simulink model "Demo_CarRealTime2D_cs"  (R2014b)
settings: Solver=ode5  SolverMode=SingleTasking  StartTime=0.0  StopTime=inf  FixedStep=1/1000  RelTol=1e-3
PreLoadFcn:
  | mbxruntime.callbacks.PreLoadFcn(bdroot);
  | check_NUTS_defined;
  | assignin('base',['model_closed_' bdroot],false);
  | addpath('../includes_AEBS');
PostLoadFcn:
  | mbxruntime.callbacks.PostLoadFcn(bdroot);
InitFcn:
  | mbxruntime.callbacks.InitFcn(bdroot);
StartFcn:
  | mbxruntime.callbacks.StartFcn(bdroot);
StopFcn:
  | mbxruntime.callbacks.StopFcn(bdroot);;
  | 
model workspace: external: MAT-File .\Demo_CarRealTime2D_cs_hws.mat (data not in the file)
undefined symbols (not defined in the file or in its folder): Driver_Demands, mbxruntime, tabledata, vicrt_initcallback, vicrt_initmexcallback, vicrt_simulationmanager, warningInitialVelocity, x0
undefined symbols (not defined in the file): Demo_CarRealTime2D_cs_007c1c37f387f47f, Demo_CarRealTime2D_cs_085a64a83ba38cec, Demo_CarRealTime2D_cs_0a7f542d3fc7ab9f, Demo_CarRealTime2D_cs_0d7c72cfaa56dff7, Demo_CarRealTime2D_cs_0de07b35068e3828, Demo_CarRealTime2D_cs_17f4d381375cce95, Demo_CarRealTime2D_cs_1db40a09b08215a9, Demo_CarRealTime2D_cs_2bfa3850c176687b, Demo_CarRealTime2D_cs_35a34f1ba6ce4a22, Demo_CarRealTime2D_cs_378cc77e08d643fb, Demo_CarRealTime2D_cs_409b5c3befba0000, Demo_CarRealTime2D_cs_42628ca5bb62d2f3, Demo_CarRealTime2D_cs_56554a2db408a7f8, Demo_CarRealTime2D_cs_59527455249d7429, Demo_CarRealTime2D_cs_5983ee1b8112afac, Demo_CarRealTime2D_cs_5b5ebcf3ed7bf8e6, Demo_CarRealTime2D_cs_63cbe7fbe16cd5d9, Demo_CarRealTime2D_cs_6e17b9adbf989abf, Demo_CarRealTime2D_cs_6f662a34e5d9a196, Demo_CarRealTime2D_cs_75c4ee8892821e19, Demo_CarRealTime2D_cs_7c64486355814be2, Demo_CarRealTime2D_cs_849809550a2230ef, Demo_CarRealTime2D_cs_87f899bcbe16d8f5, Demo_CarRealTime2D_cs_8e7b50dac25b68a2, Demo_CarRealTime2D_cs_94938e5260f139b3, Demo_CarRealTime2D_cs_983acc940698d1d1, Demo_CarRealTime2D_cs_9d554c72797f76fd, Demo_CarRealTime2D_cs_9d747ee2f15c057f, Demo_CarRealTime2D_cs_ad62a2084d31e898, Demo_CarRealTime2D_cs_b56c8c5f000d30f0, Demo_CarRealTime2D_cs_b95f1b7356e926cc, Demo_CarRealTime2D_cs_BMW_X5_1_Path_pathUniqueID, Demo_CarRealTime2D_cs_BMW_Z3_2_Dynamics_Empty_STATE_BMW_Z3_2_x0, Demo_CarRealTime2D_cs_BMW_Z3_2_Dynamics_Empty_STATE_BMW_Z3_2_y0, Demo_CarRealTime2D_cs_BMW_Z3_2_Dynamics_Empty_STATE_BMW_Z3_2_z0, Demo_CarRealTime2D_cs_BMW_Z3_Path_pathUniqueID, Demo_CarRealTime2D_cs_BMW_Z3_SpeedProfile_speedProfileUniqueID, Demo_CarRealTime2D_cs_c8847ab2e5633224, Demo_CarRealTime2D_cs_c9a0d701286b93fb, Demo_CarRealTime2D_cs_ce758cae7dd1b283, Demo_CarRealTime2D_cs_CrossingPedestrian_Path_pathUniqueID, Demo_CarRealTime2D_cs_CuttingInVehicle_Path_pathUniqueID, Demo_CarRealTime2D_cs_d901ab1c1d2e40bc, Demo_CarRealTime2D_cs_dff70430e5a00a86, Demo_CarRealTime2D_cs_ef038a4f619ad32e, Demo_CarRealTime2D_cs_Female_OverweightAni_1_Path_pathUniqueID, Demo_CarRealTime2D_cs_Ford_Fiesta_1_Path_pathUniqueID, Demo_CarRealTime2D_cs_Ford_FocusWagon_Path_pathUniqueID, Demo_CarRealTime2D_cs_Sphere_1_Dynamics_Empty_STATE_Sphere_1_x0, Demo_CarRealTime2D_cs_Sphere_1_Dynamics_Empty_STATE_Sphere_1_y0, Demo_CarRealTime2D_cs_Sphere_1_Dynamics_Empty_STATE_Sphere_1_z0, WheelL0, WheelL1, WheelR0, WheelR1
libraries: PreScanSimulinkLibrary x15, simulink x15, simulink_extras x15, PreScanUsefulBlocks x2, dspsigops x1
(part 15 of 17)

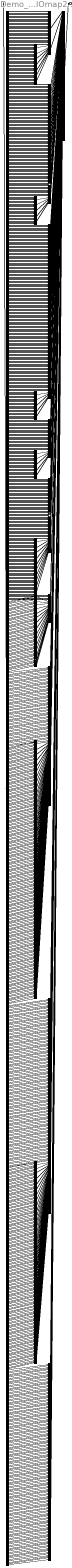
== system Demo_CarRealTime2D_cs/HostVehicle/Dynamics_UserSpecified/VI-CarRealTime/Output_Bus/IOmap2bus ==
  In : Inport
  Actual_Tread_Speed : BusCreator
  Aggregate_Force_At_Wheel : BusCreator
  Alpha : BusCreator
  Animator_Widget : BusCreator  Inputs=2
  Auxiliary_Roll_Force : BusCreator
  Auxiliary_Roll_Force_at_element : BusCreator  Inputs=2
  Auxiliary_Roll_deformation_at_element : BusCreator  Inputs=2
  Brake : BusCreator  Inputs=7
  Brake_Moment : BusCreator
  Caster_Angle : BusCreator  Inputs=2
  Chamber_Pressure : BusCreator
  Contact_Patch_Global_X : BusCreator
  Contact_Patch_Global_Y : BusCreator
  Contact_Patch_Global_Z : BusCreator
  Contact_Patch_Global_dZdX : BusCreator
  Contact_Patch_Global_dZdY : BusCreator
  Damper : BusCreator  Inputs=5
  Demux : Demux  Outputs=1108
  Drive_Moment : BusCreator
  Effective_Closing_Speed : BusCreator
  Effective_Penetration : BusCreator
  Effective_Rolling_Radius : BusCreator
  Equivalent_Tread_Speed : BusCreator
  Euler_Roll : BusCreator
  External_Friction_Scale_Factor : BusCreator
  Force_At_Bumper : BusCreator
  Force_At_Bumper1 : BusCreator
  Force_At_Damper : BusCreator
  Force_At_Spring : BusCreator
  Force_At_Wheel{,1..3} (4 alike) : BusCreator
  Force_Aux_At_Wheel : BusCreator
  Global_Omega_X : BusCreator
  Global_Omega_Y : BusCreator
  Global_Omega_Z : BusCreator
  Global_Vx : BusCreator
  Global_Vy : BusCreator
  Global_Vz : BusCreator
  Global_X : BusCreator
  Global_Y : BusCreator
  Global_Z : BusCreator
  Ground_Surface_Contact_Patch_Vx : BusCreator
  Ground_Surface_Contact_Patch_Vy : BusCreator
  Ground_Surface_Force_X : BusCreator
  Ground_Surface_Force_Y : BusCreator
  Ground_Surface_Force_Z : BusCreator
  Ground_Surface_Gyroscopic_Moment : BusCreator
  Ground_Surface_Kappa_Fy : BusCreator
  Ground_Surface_Moment_X : BusCreator
  Ground_Surface_Moment_Y : BusCreator
  Ground_Surface_Moment_Z : BusCreator
  Ground_Surface_Peak_Friction_X : BusCreator
  Ground_Surface_Peak_Friction_Y : BusCreator
  Ground_Surface_Residual_Torque : BusCreator
  Ground_Surface_Wheel_Center_Vx : BusCreator
  Gyro : BusCreator  Inputs=10
  Hook_rear : BusCreator  Inputs=18
  Hub_Carrier_Force_Global_X : BusCreator
  Hub_Carrier_Force_Global_Y : BusCreator
  Hub_Carrier_Force_Global_Z : BusCreator
  Hub_Carrier_Force_Local_X : BusCreator
  Hub_Carrier_Force_Local_Y : BusCreator
  Hub_Carrier_Force_Local_Z : BusCreator
  Hub_Carrier_Moment_Global_X : BusCreator
  Hub_Carrier_Moment_Global_Y : BusCreator
  Hub_Carrier_Moment_Global_Z : BusCreator
  Hub_Carrier_Moment_Local_X : BusCreator
  Hub_Carrier_Moment_Local_Y : BusCreator
  Hub_Carrier_Moment_Local_Z : BusCreator
  Hub_Carrier_Omega_X : BusCreator
  Hub_Carrier_Omega_Y : BusCreator
  Hub_Carrier_Omega_Z : BusCreator
  Hub_Carrier_Vx : BusCreator
  Hub_Carrier_Vy : BusCreator
  Hub_Carrier_Vz : BusCreator
  Inclination : BusCreator
  Inst_Stiff_Deflection : BusCreator
  Inst_Stiff_Force : BusCreator
  Jounce{,1..4} (5 alike) : BusCreator
  Jounce_Acceleration{,1..4} (5 alike) : BusCreator
  Jounce_Bumper : BusCreator  Inputs=5
  Jounce_Rate{,1..4} (5 alike) : BusCreator
  Kingpin_Moment : BusCreator  Inputs=1
  Kingpin_Moment1 : BusCreator  Inputs=2
  Lateral_Relaxation_Length : BusCreator
  Lateral_Slip_With_Lag : BusCreator
  Lateral_Slip_Without_Lag : BusCreator
  Loaded_Radius : BusCreator
  Locked_Damper_Moment : BusCreator
  Locked_Moment : BusCreator
  Locked_Spring_Moment : BusCreator
  Locked_Switch : BusCreator
  Lockup_Rotation : BusCreator
  Longitudinal_Relaxation_Length : BusCreator
  Longitudinal_Slip_With_Lag : BusCreator
  Longitudinal_Slip_Without_Lag : BusCreator
  Moment_Arm_Of_Fx : BusCreator
  Omega : BusCreator
  OutputBus : BusCreator  Inputs=92
  PID_CW_At_Spring : BusCreator
  PID_PH_At_Spring : BusCreator
  PID_RH_At_Spring : BusCreator
  Phi : BusCreator
  Pitch : BusCreator
  Pneumatic_Trail : BusCreator
  Psi : BusCreator
  Rebound_Bumper : BusCreator  Inputs=5
  Roll : BusCreator  Inputs=2
  Rotation : BusCreator
  Sensor : BusCreator  Inputs=16
  Side_View_Angle : BusCreator
  Spindle_Steer : BusCreator
  Spring : BusCreator  Inputs=10
  Steering_Instant_Axis_Rotation : BusCreator  Inputs=2
  Steering_System : BusCreator  Inputs=6
  Suspension : BusCreator  Inputs=14
  System : BusCreator
  System_Mass_Center : BusCreator  Inputs=13
  Theta : BusCreator
  TieRod_Force_Left : BusCreator  Inputs=3
  TieRod_Force_Right : BusCreator  Inputs=3
  Tire : BusCreator  Inputs=46
  User_Input_Contact_Patch_Global_Z_Perturbation : BusCreator
  Vehicle : BusCreator  Inputs=46
  Vehicle_States : BusCreator  Inputs=20
  Wheel : BusCreator  Inputs=37
  Yaw : BusCreator
  aero_forces : BusCreator  Inputs=24
  base_acceleration : BusCreator
  base_deformation : BusCreator
  base_velocity : BusCreator
  bul_jounce_stop_data : BusCreator  Inputs=6
  bul_rebound_stop_data : BusCreator  Inputs=6
  bur_jounce_stop_data : BusCreator  Inputs=6
  bur_rebound_stop_data : BusCreator  Inputs=6
  bus_dmp_jounce_stop_data : BusCreator  Inputs=6
  bus_ins_jounce_stop_data : BusCreator  Inputs=6
  bus_roll_dmp_jounce_stop_data : BusCreator  Inputs=6
  bus_spr_jounce_stop_data : BusCreator  Inputs=6
  chassis_accelerations : BusCreator  Inputs=6
  chassis_displacements : BusCreator  Inputs=9
  chassis_velocities : BusCreator  Inputs=6
  clutch : BusCreator  Inputs=2
  condition_sensors : BusCreator  Inputs=1
  cp_force_lateralFL : BusCreator  Inputs=3
  cp_force_lateralFR : BusCreator  Inputs=3
  cp_force_lateralRL : BusCreator  Inputs=3
  cp_force_lateralRR : BusCreator  Inputs=3
  cp_force_longitudinalFL : BusCreator  Inputs=3
  cp_force_longitudinalFR : BusCreator  Inputs=3
  cp_force_longitudinalRL : BusCreator  Inputs=3
  cp_force_longitudinalRR : BusCreator  Inputs=3
  cp_force_normalFL : BusCreator  Inputs=3
  cp_force_normalFR : BusCreator  Inputs=3
  cp_force_normalRL : BusCreator  Inputs=3
  cp_force_normalRR : BusCreator  Inputs=3
  cross_weight : BusCreator
  dal_ride_damper_data : BusCreator
  dar_ride_damper_data : BusCreator
  das_ride_damper_data : BusCreator  Inputs=6
  das_roll_damper_data : BusCreator  Inputs=8
  das_third_damper_data : BusCreator  Inputs=6
  differential_speeds : BusCreator  Inputs=6
  differential_torques : BusCreator  Inputs=6
  driver_demands : BusCreator  Inputs=7
  driving_machine_monitor : BusCreator  Inputs=9
  engine : BusCreator  Inputs=7
  fuel_consumption : BusCreator
  ges_chassis_XFORM : BusCreator  Inputs=6
  ges_hub_XFORMFL : BusCreator  Inputs=6
  ges_hub_XFORMFR : BusCreator  Inputs=6
  ges_hub_XFORMRL : BusCreator  Inputs=6
  ges_hub_XFORMRR : BusCreator  Inputs=6
  hub2cp_XFORMFL : BusCreator  Inputs=3
  hub2cp_XFORMFR : BusCreator  Inputs=3
  hub2cp_XFORMRL : BusCreator  Inputs=3
  hub2cp_XFORMRR : BusCreator  Inputs=3
  hub_center_accx : BusCreator
  hub_center_accy : BusCreator
  hub_center_accz : BusCreator
  ins_inerter_data : BusCreator  Inputs=10
  jfs_torsional_stiffness_data : BusCreator  Inputs=12
  nsl_ride_spring_data : BusCreator  Inputs=6
  nsr_ride_spring_data : BusCreator  Inputs=6
  nss_ride_spring_data : BusCreator  Inputs=10
  res_dmp_rebound_stop_data : BusCreator  Inputs=6
  res_ins_rebound_stop_data : BusCreator  Inputs=6
  res_roll_dmp_rebound_stop_data : BusCreator  Inputs=6
  res_spr_rebound_stop_data : BusCreator  Inputs=6
  rhl_front_setup_sensor_data : BusCreator  Inputs=1
  rhr_front_setup_sensor_data : BusCreator  Inputs=1
  rhs_rear_setup_sensor_data : BusCreator  Inputs=1
  til_wheel_tire_forces : BusCreator  Inputs=18
  til_wheel_tire_kinematics : BusCreator  Inputs=9
  til_wheel_tire_rolling_states : BusCreator  Inputs=9
  tir_wheel_tire_forces : BusCreator  Inputs=18
  tir_wheel_tire_kinematics : BusCreator  Inputs=9
  tir_wheel_tire_rolling_states : BusCreator  Inputs=9
  transmission : BusCreator
  ues_third_spring_data : BusCreator  Inputs=6
  upright_accelerometer : BusCreator
  wheel_angles : BusCreator  Inputs=12
  wheel_center_dispx : BusCreator
  wheel_center_dispy : BusCreator
  wheel_center_dispz : BusCreator
  whl_front_wheel_XFORM : BusCreator  Inputs=9
  whl_rear_wheel_XFORM : BusCreator  Inputs=9
  whl_twin_rear_wheel_XFORM : BusCreator  Inputs=9
  whr_front_wheel_XFORM : BusCreator  Inputs=9
  whr_rear_wheel_XFORM : BusCreator  Inputs=9
  whr_twin_rear_wheel_XFORM : BusCreator  Inputs=9
  Out : Outport
  wires:
  Demux/1108 -> cp_force_normalRR/3  "Z"
  Demux/1107 -> cp_force_normalRR/2  "Y"
  Demux/1106 -> cp_force_normalRR/1  "X"
  cp_force_normalRR/1 -> OutputBus/92  "cp_force_normalRR"
  Demux/1105 -> cp_force_lateralRR/3  "Z"
  Demux/1104 -> cp_force_lateralRR/2  "Y"
  Demux/1103 -> cp_force_lateralRR/1  "X"
  cp_force_lateralRR/1 -> OutputBus/91  "cp_force_lateralRR"
  Demux/1102 -> cp_force_longitudinalRR/3  "Z"
  Demux/1101 -> cp_force_longitudinalRR/2  "Y"
  Demux/1100 -> cp_force_longitudinalRR/1  "X"
  cp_force_longitudinalRR/1 -> OutputBus/90  "cp_force_longitudinalRR"
  Demux/1099 -> hub2cp_XFORMRR/3  "Z"
  Demux/1098 -> hub2cp_XFORMRR/2  "Y"
  Demux/1097 -> hub2cp_XFORMRR/1  "X"
  hub2cp_XFORMRR/1 -> OutputBus/89  "hub2cp_XFORMRR"
  Demux/1096 -> ges_hub_XFORMRR/6  "Phi"
  Demux/1095 -> ges_hub_XFORMRR/5  "Theta"
  Demux/1094 -> ges_hub_XFORMRR/4  "Psi"
  Demux/1093 -> ges_hub_XFORMRR/3  "Z"
  Demux/1092 -> ges_hub_XFORMRR/2  "Y"
  Demux/1091 -> ges_hub_XFORMRR/1  "X"
  ges_hub_XFORMRR/1 -> OutputBus/88  "ges_hub_XFORMRR"
  Demux/1090 -> cp_force_normalRL/3  "Z"
  Demux/1089 -> cp_force_normalRL/2  "Y"
  Demux/1088 -> cp_force_normalRL/1  "X"
  cp_force_normalRL/1 -> OutputBus/87  "cp_force_normalRL"
  Demux/1087 -> cp_force_lateralRL/3  "Z"
  Demux/1086 -> cp_force_lateralRL/2  "Y"
  Demux/1085 -> cp_force_lateralRL/1  "X"
  cp_force_lateralRL/1 -> OutputBus/86  "cp_force_lateralRL"
  Demux/1084 -> cp_force_longitudinalRL/3  "Z"
  Demux/1083 -> cp_force_longitudinalRL/2  "Y"
  Demux/1082 -> cp_force_longitudinalRL/1  "X"
  cp_force_longitudinalRL/1 -> OutputBus/85  "cp_force_longitudinalRL"
  Demux/1081 -> hub2cp_XFORMRL/3  "Z"
  Demux/1080 -> hub2cp_XFORMRL/2  "Y"
  Demux/1079 -> hub2cp_XFORMRL/1  "X"
  hub2cp_XFORMRL/1 -> OutputBus/84  "hub2cp_XFORMRL"
  Demux/1078 -> ges_hub_XFORMRL/6  "Phi"
  Demux/1077 -> ges_hub_XFORMRL/5  "Theta"
  Demux/1076 -> ges_hub_XFORMRL/4  "Psi"
  Demux/1075 -> ges_hub_XFORMRL/3  "Z"
  Demux/1074 -> ges_hub_XFORMRL/2  "Y"
  Demux/1073 -> ges_hub_XFORMRL/1  "X"
  ges_hub_XFORMRL/1 -> OutputBus/83  "ges_hub_XFORMRL"
  Demux/1072 -> cp_force_normalFR/3  "Z"
  Demux/1071 -> cp_force_normalFR/2  "Y"
  Demux/1070 -> cp_force_normalFR/1  "X"
  cp_force_normalFR/1 -> OutputBus/82  "cp_force_normalFR"
  Demux/1069 -> cp_force_lateralFR/3  "Z"
  Demux/1068 -> cp_force_lateralFR/2  "Y"
  Demux/1067 -> cp_force_lateralFR/1  "X"
  cp_force_lateralFR/1 -> OutputBus/81  "cp_force_lateralFR"
  Demux/1066 -> cp_force_longitudinalFR/3  "Z"
  Demux/1065 -> cp_force_longitudinalFR/2  "Y"
  Demux/1064 -> cp_force_longitudinalFR/1  "X"
  cp_force_longitudinalFR/1 -> OutputBus/80  "cp_force_longitudinalFR"
  Demux/1063 -> hub2cp_XFORMFR/3  "Z"
  Demux/1062 -> hub2cp_XFORMFR/2  "Y"
  Demux/1061 -> hub2cp_XFORMFR/1  "X"
  hub2cp_XFORMFR/1 -> OutputBus/79  "hub2cp_XFORMFR"
  Demux/1060 -> ges_hub_XFORMFR/6  "Phi"
  Demux/1059 -> ges_hub_XFORMFR/5  "Theta"
  Demux/1058 -> ges_hub_XFORMFR/4  "Psi"
  Demux/1057 -> ges_hub_XFORMFR/3  "Z"
  Demux/1056 -> ges_hub_XFORMFR/2  "Y"
  Demux/1055 -> ges_hub_XFORMFR/1  "X"
  ges_hub_XFORMFR/1 -> OutputBus/78  "ges_hub_XFORMFR"
  Demux/1054 -> cp_force_normalFL/3  "Z"
  Demux/1053 -> cp_force_normalFL/2  "Y"
  Demux/1052 -> cp_force_normalFL/1  "X"
  cp_force_normalFL/1 -> OutputBus/77  "cp_force_normalFL"
  Demux/1051 -> cp_force_lateralFL/3  "Z"
  Demux/1050 -> cp_force_lateralFL/2  "Y"
  Demux/1049 -> cp_force_lateralFL/1  "X"
  cp_force_lateralFL/1 -> OutputBus/76  "cp_force_lateralFL"
  Demux/1048 -> cp_force_longitudinalFL/3  "Z"
  Demux/1047 -> cp_force_longitudinalFL/2  "Y"
  Demux/1046 -> cp_force_longitudinalFL/1  "X"
  cp_force_longitudinalFL/1 -> OutputBus/75  "cp_force_longitudinalFL"
  Demux/1045 -> hub2cp_XFORMFL/3  "Z"
  Demux/1044 -> hub2cp_XFORMFL/2  "Y"
  Demux/1043 -> hub2cp_XFORMFL/1  "X"
  hub2cp_XFORMFL/1 -> OutputBus/74  "hub2cp_XFORMFL"
  Demux/1042 -> ges_hub_XFORMFL/6  "Phi"
  Demux/1041 -> ges_hub_XFORMFL/5  "Theta"
  Demux/1040 -> ges_hub_XFORMFL/4  "Psi"
  Demux/1039 -> ges_hub_XFORMFL/3  "Z"
  Demux/1038 -> ges_hub_XFORMFL/2  "Y"
  Demux/1037 -> ges_hub_XFORMFL/1  "X"
  ges_hub_XFORMFL/1 -> OutputBus/73  "ges_hub_XFORMFL"
  Demux/1036 -> Animator_Widget/2  "engine_rpm"
  Demux/1035 -> Animator_Widget/1  "longitudinal_speed"
  Animator_Widget/1 -> OutputBus/72  "Animator_Widget"
  Demux/1034 -> whr_twin_rear_wheel_XFORM/9  "Z"
  Demux/1033 -> whr_twin_rear_wheel_XFORM/8  "Y"
  Demux/1032 -> whr_twin_rear_wheel_XFORM/7  "X"
  Demux/1031 -> whr_twin_rear_wheel_XFORM/6  "Theta"
  Demux/1030 -> whr_twin_rear_wheel_XFORM/5  "Psi"
  Demux/1029 -> whr_twin_rear_wheel_XFORM/4  "Phi"
  Demux/1028 -> whr_twin_rear_wheel_XFORM/3  "FZ"
  Demux/1027 -> whr_twin_rear_wheel_XFORM/2  "FY"
  Demux/1026 -> whr_twin_rear_wheel_XFORM/1  "FX"
  whr_twin_rear_wheel_XFORM/1 -> OutputBus/71  "whr_twin_rear_wheel_XFORM"
  Demux/1025 -> whr_rear_wheel_XFORM/9  "Z"
  Demux/1024 -> whr_rear_wheel_XFORM/8  "Y"
  Demux/1023 -> whr_rear_wheel_XFORM/7  "X"
  Demux/1022 -> whr_rear_wheel_XFORM/6  "Theta"
  Demux/1021 -> whr_rear_wheel_XFORM/5  "Psi"
  Demux/1020 -> whr_rear_wheel_XFORM/4  "Phi"
  Demux/1019 -> whr_rear_wheel_XFORM/3  "FZ"
  Demux/1018 -> whr_rear_wheel_XFORM/2  "FY"
  Demux/1017 -> whr_rear_wheel_XFORM/1  "FX"
  whr_rear_wheel_XFORM/1 -> OutputBus/70  "whr_rear_wheel_XFORM"
  Demux/1016 -> whr_front_wheel_XFORM/9  "Z"
  Demux/1015 -> whr_front_wheel_XFORM/8  "Y"
  Demux/1014 -> whr_front_wheel_XFORM/7  "X"
  Demux/1013 -> whr_front_wheel_XFORM/6  "Theta"
  Demux/1012 -> whr_front_wheel_XFORM/5  "Psi"
  Demux/1011 -> whr_front_wheel_XFORM/4  "Phi"
  Demux/1010 -> whr_front_wheel_XFORM/3  "FZ"
  Demux/1009 -> whr_front_wheel_XFORM/2  "FY"
  Demux/1008 -> whr_front_wheel_XFORM/1  "FX"
  whr_front_wheel_XFORM/1 -> OutputBus/69  "whr_front_wheel_XFORM"
  Demux/1007 -> whl_twin_rear_wheel_XFORM/9  "Z"
  Demux/1006 -> whl_twin_rear_wheel_XFORM/8  "Y"
  Demux/1005 -> whl_twin_rear_wheel_XFORM/7  "X"
  Demux/1004 -> whl_twin_rear_wheel_XFORM/6  "Theta"
  Demux/1003 -> whl_twin_rear_wheel_XFORM/5  "Psi"
  Demux/1002 -> whl_twin_rear_wheel_XFORM/4  "Phi"
  Demux/1001 -> whl_twin_rear_wheel_XFORM/3  "FZ"
  Demux/1000 -> whl_twin_rear_wheel_XFORM/2  "FY"
  Demux/999 -> whl_twin_rear_wheel_XFORM/1  "FX"
  whl_twin_rear_wheel_XFORM/1 -> OutputBus/68  "whl_twin_rear_wheel_XFORM"
  Demux/998 -> whl_rear_wheel_XFORM/9  "Z"
  Demux/997 -> whl_rear_wheel_XFORM/8  "Y"
  Demux/996 -> whl_rear_wheel_XFORM/7  "X"
  Demux/995 -> whl_rear_wheel_XFORM/6  "Theta"
  Demux/994 -> whl_rear_wheel_XFORM/5  "Psi"
  Demux/993 -> whl_rear_wheel_XFORM/4  "Phi"
  Demux/992 -> whl_rear_wheel_XFORM/3  "FZ"
  Demux/991 -> whl_rear_wheel_XFORM/2  "FY"
  Demux/990 -> whl_rear_wheel_XFORM/1  "FX"
  whl_rear_wheel_XFORM/1 -> OutputBus/67  "whl_rear_wheel_XFORM"
  Demux/989 -> whl_front_wheel_XFORM/9  "Z"
  Demux/988 -> whl_front_wheel_XFORM/8  "Y"
  Demux/987 -> whl_front_wheel_XFORM/7  "X"
  Demux/986 -> whl_front_wheel_XFORM/6  "Theta"
  Demux/985 -> whl_front_wheel_XFORM/5  "Psi"
  Demux/984 -> whl_front_wheel_XFORM/4  "Phi"
  Demux/983 -> whl_front_wheel_XFORM/3  "FZ"
  Demux/982 -> whl_front_wheel_XFORM/2  "FY"
  Demux/981 -> whl_front_wheel_XFORM/1  "FX"
  whl_front_wheel_XFORM/1 -> OutputBus/66  "whl_front_wheel_XFORM"
  Demux/980 -> wheel_angles/12  "toe_R2"
  Demux/979 -> wheel_angles/11  "toe_R1"
  Demux/978 -> wheel_angles/10  "toe_L2"
  Demux/977 -> wheel_angles/9  "toe_L1"
  Demux/976 -> wheel_angles/8  "caster_R2"
  Demux/975 -> wheel_angles/7  "caster_R1"
  Demux/974 -> wheel_angles/6  "caster_L2"
  Demux/973 -> wheel_angles/5  "caster_L1"
  Demux/972 -> wheel_angles/4  "camber_R2"
  Demux/971 -> wheel_angles/3  "camber_R1"
  Demux/970 -> wheel_angles/2  "camber_L2"
  Demux/969 -> wheel_angles/1  "camber_L1"
  wheel_angles/1 -> OutputBus/65  "wheel_angles"
  Demux/968 -> Yaw/4  "R2"
  Demux/967 -> Yaw/3  "R1"
  Demux/966 -> Yaw/2  "L2"
  Demux/965 -> Yaw/1  "L1"
  Yaw/1 -> Wheel/37  "Yaw"
  Demux/964 -> wheel_center_dispz/4  "rear_right"
  Demux/963 -> wheel_center_dispz/3  "rear_left"
  Demux/962 -> wheel_center_dispz/2  "front_right"
  Demux/961 -> wheel_center_dispz/1  "front_left"
  wheel_center_dispz/1 -> Wheel/36  "wheel_center_dispz"
  Demux/960 -> wheel_center_dispy/4  "rear_right"
  Demux/959 -> wheel_center_dispy/3  "rear_left"
  Demux/958 -> wheel_center_dispy/2  "front_right"
  Demux/957 -> wheel_center_dispy/1  "front_left"
  wheel_center_dispy/1 -> Wheel/35  "wheel_center_dispy"
  Demux/956 -> wheel_center_dispx/4  "rear_right"
  Demux/955 -> wheel_center_dispx/3  "rear_left"
  Demux/954 -> wheel_center_dispx/2  "front_right"
  Demux/953 -> wheel_center_dispx/1  "front_left"
  wheel_center_dispx/1 -> Wheel/34  "wheel_center_dispx"
  Demux/952 -> Theta/4  "R2"
  Demux/951 -> Theta/3  "R1"
  Demux/950 -> Theta/2  "L2"
  Demux/949 -> Theta/1  "L1"
  Theta/1 -> Wheel/33  "Theta"
  Demux/948 -> Spindle_Steer/4  "R2"
  Demux/947 -> Spindle_Steer/3  "R1"
  Demux/946 -> Spindle_Steer/2  "L2"
  Demux/945 -> Spindle_Steer/1  "L1"
  Spindle_Steer/1 -> Wheel/32  "Spindle_Steer"
  Demux/944 -> Side_View_Angle/4  "R2"
  Demux/943 -> Side_View_Angle/3  "R1"
  Demux/942 -> Side_View_Angle/2  "L2"
  Demux/941 -> Side_View_Angle/1  "L1"
  Side_View_Angle/1 -> Wheel/31  "Side_View_Angle"
  Demux/940 -> Rotation/4  "R2"
  Demux/939 -> Rotation/3  "R1"
  Demux/938 -> Rotation/2  "L2"
  Demux/937 -> Rotation/1  "L1"
  Rotation/1 -> Wheel/30  "Rotation"
  Demux/936 -> Psi/4  "R2"
  Demux/935 -> Psi/3  "R1"
  Demux/934 -> Psi/2  "L2"
  Demux/933 -> Psi/1  "L1"
  Psi/1 -> Wheel/29  "Psi"
  Demux/932 -> Pitch/4  "R2"
  Demux/931 -> Pitch/3  "R1"
  Demux/930 -> Pitch/2  "L2"
  Demux/929 -> Pitch/1  "L1"
  Pitch/1 -> Wheel/28  "Pitch"
  Demux/928 -> Phi/4  "R2"
  Demux/927 -> Phi/3  "R1"
  Demux/926 -> Phi/2  "L2"
  Demux/925 -> Phi/1  "L1"
  Phi/1 -> Wheel/27  "Phi"
  Demux/924 -> Omega/4  "R2"
  Demux/923 -> Omega/3  "R1"
  Demux/922 -> Omega/2  "L2"
  Demux/921 -> Omega/1  "L1"
  Omega/1 -> Wheel/26  "Omega"
  Demux/920 -> Kingpin_Moment1/2  "R1"
  Demux/919 -> Kingpin_Moment1/1  "L1"
  Kingpin_Moment1/1 -> Wheel/25  "Kingpin_Moment"
  Demux/918 -> Inclination/4  "R2"
  Demux/917 -> Inclination/3  "R1"
  Demux/916 -> Inclination/2  "L2"
  Demux/915 -> Inclination/1  "L1"
  Inclination/1 -> Wheel/24  "Inclination"
  Demux/914 -> hub_center_accz/4  "rear_right"
  Demux/913 -> hub_center_accz/3  "rear_left"
  Demux/912 -> hub_center_accz/2  "front_right"
  Demux/911 -> hub_center_accz/1  "front_left"
  hub_center_accz/1 -> Wheel/23  "hub_center_accz"
  Demux/910 -> hub_center_accy/4  "rear_right"
  Demux/909 -> hub_center_accy/3  "rear_left"
  Demux/908 -> hub_center_accy/2  "front_right"
  Demux/907 -> hub_center_accy/1  "front_left"
  hub_center_accy/1 -> Wheel/22  "hub_center_accy"
  Demux/906 -> hub_center_accx/4  "rear_right"
  Demux/905 -> hub_center_accx/3  "rear_left"
  Demux/904 -> hub_center_accx/2  "front_right"
  Demux/903 -> hub_center_accx/1  "front_left"
  hub_center_accx/1 -> Wheel/21  "hub_center_accx"
  Demux/902 -> Hub_Carrier_Vz/4  "R2"
  Demux/901 -> Hub_Carrier_Vz/3  "R1"
  Demux/900 -> Hub_Carrier_Vz/2  "L2"
  Demux/899 -> Hub_Carrier_Vz/1  "L1"
  Hub_Carrier_Vz/1 -> Wheel/20  "Hub_Carrier_Vz"
  Demux/898 -> Hub_Carrier_Vy/4  "R2"
  Demux/897 -> Hub_Carrier_Vy/3  "R1"
  Demux/896 -> Hub_Carrier_Vy/2  "L2"
  Demux/895 -> Hub_Carrier_Vy/1  "L1"
  Hub_Carrier_Vy/1 -> Wheel/19  "Hub_Carrier_Vy"
  Demux/894 -> Hub_Carrier_Vx/4  "R2"
  Demux/893 -> Hub_Carrier_Vx/3  "R1"
  Demux/892 -> Hub_Carrier_Vx/2  "L2"
  Demux/891 -> Hub_Carrier_Vx/1  "L1"
  Hub_Carrier_Vx/1 -> Wheel/18  "Hub_Carrier_Vx"
  Demux/890 -> Hub_Carrier_Omega_Z/4  "R2"
  Demux/889 -> Hub_Carrier_Omega_Z/3  "R1"
  Demux/888 -> Hub_Carrier_Omega_Z/2  "L2"
  Demux/887 -> Hub_Carrier_Omega_Z/1  "L1"
  Hub_Carrier_Omega_Z/1 -> Wheel/17  "Hub_Carrier_Omega_Z"
  Demux/886 -> Hub_Carrier_Omega_Y/4  "R2"
  Demux/885 -> Hub_Carrier_Omega_Y/3  "R1"
  Demux/884 -> Hub_Carrier_Omega_Y/2  "L2"
  Demux/883 -> Hub_Carrier_Omega_Y/1  "L1"
  Hub_Carrier_Omega_Y/1 -> Wheel/16  "Hub_Carrier_Omega_Y"
  Demux/882 -> Hub_Carrier_Omega_X/4  "R2"
  Demux/881 -> Hub_Carrier_Omega_X/3  "R1"
  Demux/880 -> Hub_Carrier_Omega_X/2  "L2"
  Demux/879 -> Hub_Carrier_Omega_X/1  "L1"
  Hub_Carrier_Omega_X/1 -> Wheel/15  "Hub_Carrier_Omega_X"
  Demux/878 -> Ground_Surface_Wheel_Center_Vx/4  "R2"
  Demux/877 -> Ground_Surface_Wheel_Center_Vx/3  "R1"
  Demux/876 -> Ground_Surface_Wheel_Center_Vx/2  "L2"
  Demux/875 -> Ground_Surface_Wheel_Center_Vx/1  "L1"
  Ground_Surface_Wheel_Center_Vx/1 -> Wheel/14  "Ground_Surface_Wheel_Center_Vx"
  Demux/874 -> Global_Z/4  "R2"
  Demux/873 -> Global_Z/3  "R1"
  Demux/872 -> Global_Z/2  "L2"
  Demux/871 -> Global_Z/1  "L1"
  Global_Z/1 -> Wheel/13  "Global_Z"
  Demux/870 -> Global_Y/4  "R2"
  Demux/869 -> Global_Y/3  "R1"
  Demux/868 -> Global_Y/2  "L2"
  Demux/867 -> Global_Y/1  "L1"
  Global_Y/1 -> Wheel/12  "Global_Y"
  Demux/866 -> Global_X/4  "R2"
  Demux/865 -> Global_X/3  "R1"
  Demux/864 -> Global_X/2  "L2"
  Demux/863 -> Global_X/1  "L1"
  Global_X/1 -> Wheel/11  "Global_X"
  Demux/862 -> Global_Vz/4  "R2"
  Demux/861 -> Global_Vz/3  "R1"
  Demux/860 -> Global_Vz/2  "L2"
  Demux/859 -> Global_Vz/1  "L1"
  Global_Vz/1 -> Wheel/10  "Global_Vz"
  Demux/858 -> Global_Vy/4  "R2"
  Demux/857 -> Global_Vy/3  "R1"
  Demux/856 -> Global_Vy/2  "L2"
  Demux/855 -> Global_Vy/1  "L1"
  Global_Vy/1 -> Wheel/9  "Global_Vy"
  Demux/854 -> Global_Vx/4  "R2"
  Demux/853 -> Global_Vx/3  "R1"
  Demux/852 -> Global_Vx/2  "L2"
  Demux/851 -> Global_Vx/1  "L1"
  Global_Vx/1 -> Wheel/8  "Global_Vx"
  Demux/850 -> Global_Omega_Z/4  "R2"
  Demux/849 -> Global_Omega_Z/3  "R1"
  Demux/848 -> Global_Omega_Z/2  "L2"
  Demux/847 -> Global_Omega_Z/1  "L1"
  Global_Omega_Z/1 -> Wheel/7  "Global_Omega_Z"
  Demux/846 -> Global_Omega_Y/4  "R2"
  Demux/845 -> Global_Omega_Y/3  "R1"
  Demux/844 -> Global_Omega_Y/2  "L2"
  Demux/843 -> Global_Omega_Y/1  "L1"
  Global_Omega_Y/1 -> Wheel/6  "Global_Omega_Y"
  Demux/842 -> Global_Omega_X/4  "R2"
  Demux/841 -> Global_Omega_X/3  "R1"
  Demux/840 -> Global_Omega_X/2  "L2"
  Demux/839 -> Global_Omega_X/1  "L1"
  Global_Omega_X/1 -> Wheel/5  "Global_Omega_X"
  Demux/838 -> Euler_Roll/4  "R2"
  Demux/837 -> Euler_Roll/3  "R1"
  Demux/836 -> Euler_Roll/2  "L2"
  Demux/835 -> Euler_Roll/1  "L1"
  Euler_Roll/1 -> Wheel/4  "Euler_Roll"
  Demux/834 -> Drive_Moment/4  "R2"
  Demux/833 -> Drive_Moment/3  "R1"
  Demux/832 -> Drive_Moment/2  "L2"
  Demux/831 -> Drive_Moment/1  "L1"
  Drive_Moment/1 -> Wheel/3  "Drive_Moment"
  Demux/830 -> Caster_Angle/2  "right"
  Demux/829 -> Caster_Angle/1  "left"
  Caster_Angle/1 -> Wheel/2  "Caster_Angle"
  Demux/828 -> Alpha/4  "R2"
  Demux/827 -> Alpha/3  "R1"
  Demux/826 -> Alpha/2  "L2"
  Demux/825 -> Alpha/1  "L1"
  Alpha/1 -> Wheel/1  "Alpha"
  Wheel/1 -> OutputBus/64  "Wheel"
  Demux/824 -> Vehicle_States/20  "yaw_angular_vel_wrt_road"
  Demux/823 -> Vehicle_States/19  "yaw_angular_acc_wrt_road"
  Demux/822 -> Vehicle_States/18  "yaw_angle"
  Demux/821 -> Vehicle_States/17  "vertical_vel_wrt_road"
  Demux/820 -> Vehicle_States/16  "vertical_disp"
  Demux/819 -> Vehicle_States/15  "vertical_acc_wrt_road"
  Demux/818 -> Vehicle_States/14  "side_slip"
  Demux/817 -> Vehicle_States/13  "roll_angular_vel_wrt_road"
  Demux/816 -> Vehicle_States/12  "roll_angular_acc_wrt_road"
  Demux/815 -> Vehicle_States/11  "roll_angle"
  Demux/814 -> Vehicle_States/10  "pitch_angular_vel_wrt_road"
  Demux/813 -> Vehicle_States/9  "pitch_angular_acc_wrt_road"
  Demux/812 -> Vehicle_States/8  "pitch_angle"
  Demux/811 -> Vehicle_States/7  "longitudinal_vel_wrt_road"
  Demux/810 -> Vehicle_States/6  "longitudinal_disp"
  Demux/809 -> Vehicle_States/5  "longitudinal_acc_wrt_road"
  Demux/808 -> Vehicle_States/4  "lateral_vel_wrt_road"
  Demux/807 -> Vehicle_States/3  "lateral_disp"
  Demux/806 -> Vehicle_States/2  "lateral_acc_wrt_road"
  Demux/805 -> Vehicle_States/1  "horizontal_vel_wrt_road"
  Vehicle_States/1 -> OutputBus/63  "Vehicle_States"
  Demux/804 -> Vehicle/46  "Yaw"
  Demux/803 -> Vehicle/45  "Understeer_Stability_Factor"
  Demux/802 -> Vehicle/44  "Understeer_Gradient"
  Demux/801 -> Vehicle/43  "Side_Slip_Angle_Rate"
  Demux/800 -> Vehicle/42  "Side_Slip_Angle"
  Demux/799 -> Vehicle/41  "Pitch"
  Demux/798 -> Vehicle/40  "Origin_Global_Z_wrt_road_mk"
  Demux/797 -> Vehicle/39  "Origin_Global_Z"
  Demux/796 -> Vehicle/38  "Origin_Global_Y"
  Demux/795 -> Vehicle/37  "Origin_Global_X"
  Demux/794 -> Vehicle/36  "Origin_Distance_Traveled"
  Demux/793 -> Vehicle/35  "Inclination_Roll"
  Demux/792 -> Vehicle/34  "Global_Omega_Z"
  Demux/791 -> Vehicle/33  "Global_Omega_Y"
  Demux/790 -> Vehicle/32  "Global_Omega_X"
  Demux/789 -> Vehicle/31  "Global_Alpha_Z"
  Demux/788 -> Vehicle/30  "Global_Alpha_Y"
  Demux/787 -> Vehicle/29  "Global_Alpha_X"
  Demux/786 -> Vehicle/28  "front_ride_height_at_center_point"
  Demux/785 -> Vehicle/27  "Euler_Roll"
  Demux/784 -> Vehicle/26  "cross_weight_PID"
  Demux/783 -> Vehicle/25  "CM_Tracking_Vy"
  Demux/782 -> Vehicle/24  "CM_Tracking_Vx"
  Demux/781 -> Vehicle/23  "CM_Tracking_Ay"
  Demux/780 -> Vehicle/22  "CM_Tracking_Ax"
  Demux/779 -> Vehicle/21  "CM_Global_Z"
  Demux/778 -> Vehicle/20  "CM_Global_Y"
  Demux/777 -> Vehicle/19  "CM_Global_X"
  Demux/776 -> Vehicle/18  "CM_Global_Vy"
  Demux/775 -> Vehicle/17  "CM_Global_Vx"
  Demux/774 -> Vehicle/16  "CM_Global_Ay"
  Demux/773 -> Vehicle/15  "CM_Global_Ax"
  Demux/772 -> Vehicle/14  "CM_Global_And_Tracking_Vz"
  Demux/771 -> Vehicle/13  "CM_Global_And_Tracking_Az"
  Demux/770 -> Vehicle/12  "CM_Body_Fixed_Vz"
  Demux/769 -> Vehicle/11  "CM_Body_Fixed_Vy"
  Demux/768 -> Vehicle/10  "CM_Body_Fixed_Vx"
  Demux/767 -> Vehicle/9  "CM_Body_Fixed_Az"
  Demux/766 -> Vehicle/8  "CM_Body_Fixed_Ay"
  Demux/765 -> Vehicle/7  "CM_Body_Fixed_Ax"
  Demux/764 -> Vehicle/6  "Body_Fixed_Omega_Z"
  Demux/763 -> Vehicle/5  "Body_Fixed_Omega_Y"
  Demux/762 -> Vehicle/4  "Body_Fixed_Omega_X"
  Demux/761 -> Vehicle/3  "Body_Fixed_Alpha_Z"
  Demux/760 -> Vehicle/2  "Body_Fixed_Alpha_Y"
  Demux/759 -> Vehicle/1  "Body_Fixed_Alpha_X"
  Vehicle/1 -> OutputBus/62  "Vehicle"
  Demux/758 -> upright_accelerometer/4  "Z_right_rear"
  Demux/757 -> upright_accelerometer/3  "Z_right_front"
  Demux/756 -> upright_accelerometer/2  "Z_left_rear"
  Demux/755 -> upright_accelerometer/1  "Z_left_front"
  upright_accelerometer/1 -> OutputBus/61  "upright_accelerometer"
  Demux/754 -> ues_third_spring_data/6  "velocity_rear"
  Demux/753 -> ues_third_spring_data/5  "velocity_front"
  Demux/752 -> ues_third_spring_data/4  "force_rear"
  Demux/751 -> ues_third_spring_data/3  "force_front"
  Demux/750 -> ues_third_spring_data/2  "displacement_rear"
  Demux/749 -> ues_third_spring_data/1  "displacement_front"
  ues_third_spring_data/1 -> OutputBus/60  "ues_third_spring_data"
  Demux/748 -> transmission/4  "ratio"
  Demux/747 -> transmission/3  "output_rpm"
  Demux/746 -> transmission/2  "input_rpm"
  Demux/745 -> transmission/1  "gear"
  transmission/1 -> OutputBus/59  "transmission"
  Demux/744 -> tir_wheel_tire_rolling_states/9  "rolling_radius_twin_rear"
  Demux/743 -> tir_wheel_tire_rolling_states/8  "rolling_radius_rear"
  Demux/742 -> tir_wheel_tire_rolling_states/7  "rolling_radius_front"
  Demux/741 -> tir_wheel_tire_rolling_states/6  "omega_free_twin_rear"
  Demux/740 -> tir_wheel_tire_rolling_states/5  "omega_free_rear"
  Demux/739 -> tir_wheel_tire_rolling_states/4  "omega_free_front"
  Demux/738 -> tir_wheel_tire_rolling_states/3  "omega_actual_twin_rear"
  Demux/737 -> tir_wheel_tire_rolling_states/2  "omega_actual_rear"
  Demux/736 -> tir_wheel_tire_rolling_states/1  "omega_actual_front"
  tir_wheel_tire_rolling_states/1 -> OutputBus/58  "tir_wheel_tire_rolling_states"
  Demux/735 -> tir_wheel_tire_kinematics/9  "longitudinal_slip_twin_rear"
  Demux/734 -> tir_wheel_tire_kinematics/8  "longitudinal_slip_rear"
  Demux/733 -> tir_wheel_tire_kinematics/7  "longitudinal_slip_front"
  Demux/732 -> tir_wheel_tire_kinematics/6  "lateral_slip_twin_rear"
  Demux/731 -> tir_wheel_tire_kinematics/5  "lateral_slip_rear"
  Demux/730 -> tir_wheel_tire_kinematics/4  "lateral_slip_front"
  Demux/729 -> tir_wheel_tire_kinematics/3  "inclination_angle_twin_rear"
  Demux/728 -> tir_wheel_tire_kinematics/2  "inclination_angle_rear"
  Demux/727 -> tir_wheel_tire_kinematics/1  "inclination_angle_front"
  tir_wheel_tire_kinematics/1 -> OutputBus/57  "tir_wheel_tire_kinematics"
  Demux/726 -> tir_wheel_tire_forces/18  "rolling_resistance_twin_rear"
  Demux/725 -> tir_wheel_tire_forces/17  "rolling_resistance_rear"
  Demux/724 -> tir_wheel_tire_forces/16  "rolling_resistance_front"
  Demux/723 -> tir_wheel_tire_forces/15  "overturning_moment_twin_rear"
  Demux/722 -> tir_wheel_tire_forces/14  "overturning_moment_rear"
  Demux/721 -> tir_wheel_tire_forces/13  "overturning_moment_front"
  Demux/720 -> tir_wheel_tire_forces/12  "normal_twin_rear"
  Demux/719 -> tir_wheel_tire_forces/11  "normal_rear"
  Demux/718 -> tir_wheel_tire_forces/10  "normal_front"
  Demux/717 -> tir_wheel_tire_forces/9  "longitudinal_twin_rear"
  Demux/716 -> tir_wheel_tire_forces/8  "longitudinal_rear"
  Demux/715 -> tir_wheel_tire_forces/7  "longitudinal_front"
  Demux/714 -> tir_wheel_tire_forces/6  "lateral_twin_rear"
  Demux/713 -> tir_wheel_tire_forces/5  "lateral_rear"
  Demux/712 -> tir_wheel_tire_forces/4  "lateral_front"
  Demux/711 -> tir_wheel_tire_forces/3  "aligning_torque_twin_rear"
  Demux/710 -> tir_wheel_tire_forces/2  "aligning_torque_rear"
  Demux/709 -> tir_wheel_tire_forces/1  "aligning_torque_front"
  tir_wheel_tire_forces/1 -> OutputBus/56  "tir_wheel_tire_forces"
  Demux/708 -> User_Input_Contact_Patch_Global_Z_Perturbation/4  "R2"
  Demux/707 -> User_Input_Contact_Patch_Global_Z_Perturbation/3  "R1"
  Demux/706 -> User_Input_Contact_Patch_Global_Z_Perturbation/2  "L2"
  Demux/705 -> User_Input_Contact_Patch_Global_Z_Perturbation/1  "L1"
  User_Input_Contact_Patch_Global_Z_Perturbation/1 -> Tire/46  "User_Input_Contact_Patch_Global_Z_Perturbation"
  Demux/704 -> Pneumatic_Trail/4  "R2"
  Demux/703 -> Pneumatic_Trail/3  "R1"
  Demux/702 -> Pneumatic_Trail/2  "L2"
  Demux/701 -> Pneumatic_Trail/1  "L1"
  Pneumatic_Trail/1 -> Tire/45  "Pneumatic_Trail"
  Demux/700 -> Moment_Arm_Of_Fx/4  "R2"
  Demux/699 -> Moment_Arm_Of_Fx/3  "R1"
  Demux/698 -> Moment_Arm_Of_Fx/2  "L2"
  Demux/697 -> Moment_Arm_Of_Fx/1  "L1"
  Moment_Arm_Of_Fx/1 -> Tire/44  "Moment_Arm_Of_Fx"
  Demux/696 -> Longitudinal_Slip_With_Lag/4  "R2"
  Demux/695 -> Longitudinal_Slip_With_Lag/3  "R1"
  Demux/694 -> Longitudinal_Slip_With_Lag/2  "L2"
  Demux/693 -> Longitudinal_Slip_With_Lag/1  "L1"
  Longitudinal_Slip_With_Lag/1 -> Tire/43  "Longitudinal_Slip_With_Lag"
  Demux/692 -> Longitudinal_Slip_Without_Lag/4  "R2"
  Demux/691 -> Longitudinal_Slip_Without_Lag/3  "R1"
  Demux/690 -> Longitudinal_Slip_Without_Lag/2  "L2"
  Demux/689 -> Longitudinal_Slip_Without_Lag/1  "L1"
  Longitudinal_Slip_Without_Lag/1 -> Tire/42  "Longitudinal_Slip_Without_Lag"
  Demux/688 -> Longitudinal_Relaxation_Length/4  "R2"
  Demux/687 -> Longitudinal_Relaxation_Length/3  "R1"
  Demux/686 -> Longitudinal_Relaxation_Length/2  "L2"
  Demux/685 -> Longitudinal_Relaxation_Length/1  "L1"
  Longitudinal_Relaxation_Length/1 -> Tire/41  "Longitudinal_Relaxation_Length"
  Demux/684 -> Loaded_Radius/4  "R2"
  Demux/683 -> Loaded_Radius/3  "R1"
  Demux/682 -> Loaded_Radius/2  "L2"
  Demux/681 -> Loaded_Radius/1  "L1"
  Loaded_Radius/1 -> Tire/40  "Loaded_Radius"
  Demux/680 -> Lateral_Slip_With_Lag/4  "R2"
  Demux/679 -> Lateral_Slip_With_Lag/3  "R1"
  Demux/678 -> Lateral_Slip_With_Lag/2  "L2"
  Demux/677 -> Lateral_Slip_With_Lag/1  "L1"
  Lateral_Slip_With_Lag/1 -> Tire/39  "Lateral_Slip_With_Lag"
  Demux/676 -> Lateral_Slip_Without_Lag/4  "R2"
  Demux/675 -> Lateral_Slip_Without_Lag/3  "R1"
  Demux/674 -> Lateral_Slip_Without_Lag/2  "L2"
  Demux/673 -> Lateral_Slip_Without_Lag/1  "L1"
  Lateral_Slip_Without_Lag/1 -> Tire/38  "Lateral_Slip_Without_Lag"
  Demux/672 -> Lateral_Relaxation_Length/4  "R2"
  Demux/671 -> Lateral_Relaxation_Length/3  "R1"
  Demux/670 -> Lateral_Relaxation_Length/2  "L2"
  Demux/669 -> Lateral_Relaxation_Length/1  "L1"
  Lateral_Relaxation_Length/1 -> Tire/37  "Lateral_Relaxation_Length"
  Demux/668 -> Hub_Carrier_Moment_Local_Z/4  "R2"
  Demux/667 -> Hub_Carrier_Moment_Local_Z/3  "R1"
  Demux/666 -> Hub_Carrier_Moment_Local_Z/2  "L2"
  Demux/665 -> Hub_Carrier_Moment_Local_Z/1  "L1"
  Hub_Carrier_Moment_Local_Z/1 -> Tire/36  "Hub_Carrier_Moment_Local_Z"
  Demux/664 -> Hub_Carrier_Moment_Local_Y/4  "R2"
  Demux/663 -> Hub_Carrier_Moment_Local_Y/3  "R1"
  Demux/662 -> Hub_Carrier_Moment_Local_Y/2  "L2"
  Demux/661 -> Hub_Carrier_Moment_Local_Y/1  "L1"
  Hub_Carrier_Moment_Local_Y/1 -> Tire/35  "Hub_Carrier_Moment_Local_Y"
  Demux/660 -> Hub_Carrier_Moment_Local_X/4  "R2"
  Demux/659 -> Hub_Carrier_Moment_Local_X/3  "R1"
  Demux/658 -> Hub_Carrier_Moment_Local_X/2  "L2"
  Demux/657 -> Hub_Carrier_Moment_Local_X/1  "L1"
  Hub_Carrier_Moment_Local_X/1 -> Tire/34  "Hub_Carrier_Moment_Local_X"
  Demux/656 -> Hub_Carrier_Moment_Global_Z/4  "R2"
  Demux/655 -> Hub_Carrier_Moment_Global_Z/3  "R1"
  Demux/654 -> Hub_Carrier_Moment_Global_Z/2  "L2"
  Demux/653 -> Hub_Carrier_Moment_Global_Z/1  "L1"
  Hub_Carrier_Moment_Global_Z/1 -> Tire/33  "Hub_Carrier_Moment_Global_Z"
  Demux/652 -> Hub_Carrier_Moment_Global_Y/4  "R2"
  Demux/651 -> Hub_Carrier_Moment_Global_Y/3  "R1"
  Demux/650 -> Hub_Carrier_Moment_Global_Y/2  "L2"
  Demux/649 -> Hub_Carrier_Moment_Global_Y/1  "L1"
  Hub_Carrier_Moment_Global_Y/1 -> Tire/32  "Hub_Carrier_Moment_Global_Y"
  Demux/648 -> Hub_Carrier_Moment_Global_X/4  "R2"
  Demux/647 -> Hub_Carrier_Moment_Global_X/3  "R1"
  Demux/646 -> Hub_Carrier_Moment_Global_X/2  "L2"
  Demux/645 -> Hub_Carrier_Moment_Global_X/1  "L1"
  Hub_Carrier_Moment_Global_X/1 -> Tire/31  "Hub_Carrier_Moment_Global_X"
  Demux/644 -> Hub_Carrier_Force_Local_Z/4  "R2"
  Demux/643 -> Hub_Carrier_Force_Local_Z/3  "R1"
  Demux/642 -> Hub_Carrier_Force_Local_Z/2  "L2"
  Demux/641 -> Hub_Carrier_Force_Local_Z/1  "L1"
  Hub_Carrier_Force_Local_Z/1 -> Tire/30  "Hub_Carrier_Force_Local_Z"
  Demux/640 -> Hub_Carrier_Force_Local_Y/4  "R2"
  Demux/639 -> Hub_Carrier_Force_Local_Y/3  "R1"
  Demux/638 -> Hub_Carrier_Force_Local_Y/2  "L2"
  Demux/637 -> Hub_Carrier_Force_Local_Y/1  "L1"
  Hub_Carrier_Force_Local_Y/1 -> Tire/29  "Hub_Carrier_Force_Local_Y"
  Demux/636 -> Hub_Carrier_Force_Local_X/4  "R2"
  Demux/635 -> Hub_Carrier_Force_Local_X/3  "R1"
  Demux/634 -> Hub_Carrier_Force_Local_X/2  "L2"
  Demux/633 -> Hub_Carrier_Force_Local_X/1  "L1"
  Hub_Carrier_Force_Local_X/1 -> Tire/28  "Hub_Carrier_Force_Local_X"
  Demux/632 -> Hub_Carrier_Force_Global_Z/4  "R2"
  Demux/631 -> Hub_Carrier_Force_Global_Z/3  "R1"
  Demux/630 -> Hub_Carrier_Force_Global_Z/2  "L2"
  Demux/629 -> Hub_Carrier_Force_Global_Z/1  "L1"
  Hub_Carrier_Force_Global_Z/1 -> Tire/27  "Hub_Carrier_Force_Global_Z"
  Demux/628 -> Hub_Carrier_Force_Global_Y/4  "R2"
  Demux/627 -> Hub_Carrier_Force_Global_Y/3  "R1"
  Demux/626 -> Hub_Carrier_Force_Global_Y/2  "L2"
  Demux/625 -> Hub_Carrier_Force_Global_Y/1  "L1"
  Hub_Carrier_Force_Global_Y/1 -> Tire/26  "Hub_Carrier_Force_Global_Y"
  Demux/624 -> Hub_Carrier_Force_Global_X/4  "R2"
  Demux/623 -> Hub_Carrier_Force_Global_X/3  "R1"
  Demux/622 -> Hub_Carrier_Force_Global_X/2  "L2"
  Demux/621 -> Hub_Carrier_Force_Global_X/1  "L1"
  Hub_Carrier_Force_Global_X/1 -> Tire/25  "Hub_Carrier_Force_Global_X"
  Demux/620 -> Ground_Surface_Residual_Torque/4  "R2"
  Demux/619 -> Ground_Surface_Residual_Torque/3  "R1"
  Demux/618 -> Ground_Surface_Residual_Torque/2  "L2"
  Demux/617 -> Ground_Surface_Residual_Torque/1  "L1"
  Ground_Surface_Residual_Torque/1 -> Tire/24  "Ground_Surface_Residual_Torque"
  Demux/616 -> Ground_Surface_Peak_Friction_Y/4  "R2"
  Demux/615 -> Ground_Surface_Peak_Friction_Y/3  "R1"
  Demux/614 -> Ground_Surface_Peak_Friction_Y/2  "L2"
  Demux/613 -> Ground_Surface_Peak_Friction_Y/1  "L1"
  Ground_Surface_Peak_Friction_Y/1 -> Tire/23  "Ground_Surface_Peak_Friction_Y"
  Demux/612 -> Ground_Surface_Peak_Friction_X/4  "R2"
  Demux/611 -> Ground_Surface_Peak_Friction_X/3  "R1"
  Demux/610 -> Ground_Surface_Peak_Friction_X/2  "L2"
  Demux/609 -> Ground_Surface_Peak_Friction_X/1  "L1"
  Ground_Surface_Peak_Friction_X/1 -> Tire/22  "Ground_Surface_Peak_Friction_X"
  Demux/608 -> Ground_Surface_Moment_Z/4  "R2"
  Demux/607 -> Ground_Surface_Moment_Z/3  "R1"
  Demux/606 -> Ground_Surface_Moment_Z/2  "L2"
  Demux/605 -> Ground_Surface_Moment_Z/1  "L1"
  Ground_Surface_Moment_Z/1 -> Tire/21  "Ground_Surface_Moment_Z"
  Demux/604 -> Ground_Surface_Moment_Y/4  "R2"
  Demux/603 -> Ground_Surface_Moment_Y/3  "R1"
  Demux/602 -> Ground_Surface_Moment_Y/2  "L2"
  Demux/601 -> Ground_Surface_Moment_Y/1  "L1"
  Ground_Surface_Moment_Y/1 -> Tire/20  "Ground_Surface_Moment_Y"
  Demux/600 -> Ground_Surface_Moment_X/4  "R2"
  Demux/599 -> Ground_Surface_Moment_X/3  "R1"
  Demux/598 -> Ground_Surface_Moment_X/2  "L2"
  Demux/597 -> Ground_Surface_Moment_X/1  "L1"
  Ground_Surface_Moment_X/1 -> Tire/19  "Ground_Surface_Moment_X"
  Demux/596 -> Ground_Surface_Kappa_Fy/4  "R2"
  Demux/595 -> Ground_Surface_Kappa_Fy/3  "R1"
  Demux/594 -> Ground_Surface_Kappa_Fy/2  "L2"
  Demux/593 -> Ground_Surface_Kappa_Fy/1  "L1"
  Ground_Surface_Kappa_Fy/1 -> Tire/18  "Ground_Surface_Kappa_Fy"
  Demux/592 -> Ground_Surface_Gyroscopic_Moment/4  "R2"
  Demux/591 -> Ground_Surface_Gyroscopic_Moment/3  "R1"
  Demux/590 -> Ground_Surface_Gyroscopic_Moment/2  "L2"
  Demux/589 -> Ground_Surface_Gyroscopic_Moment/1  "L1"
  Ground_Surface_Gyroscopic_Moment/1 -> Tire/17  "Ground_Surface_Gyroscopic_Moment"
  Demux/588 -> Ground_Surface_Force_Z/4  "R2"
  Demux/587 -> Ground_Surface_Force_Z/3  "R1"
  Demux/586 -> Ground_Surface_Force_Z/2  "L2"
  Demux/585 -> Ground_Surface_Force_Z/1  "L1"
  Ground_Surface_Force_Z/1 -> Tire/16  "Ground_Surface_Force_Z"
  Demux/584 -> Ground_Surface_Force_Y/4  "R2"
  Demux/583 -> Ground_Surface_Force_Y/3  "R1"
  Demux/582 -> Ground_Surface_Force_Y/2  "L2"
  Demux/581 -> Ground_Surface_Force_Y/1  "L1"
  Ground_Surface_Force_Y/1 -> Tire/15  "Ground_Surface_Force_Y"
  Demux/580 -> Ground_Surface_Force_X/4  "R2"
  Demux/579 -> Ground_Surface_Force_X/3  "R1"
  Demux/578 -> Ground_Surface_Force_X/2  "L2"
  Demux/577 -> Ground_Surface_Force_X/1  "L1"
  Ground_Surface_Force_X/1 -> Tire/14  "Ground_Surface_Force_X"
  Demux/576 -> Ground_Surface_Contact_Patch_Vy/4  "R2"
  Demux/575 -> Ground_Surface_Contact_Patch_Vy/3  "R1"
  Demux/574 -> Ground_Surface_Contact_Patch_Vy/2  "L2"
  Demux/573 -> Ground_Surface_Contact_Patch_Vy/1  "L1"
  Ground_Surface_Contact_Patch_Vy/1 -> Tire/13  "Ground_Surface_Contact_Patch_Vy"
  Demux/572 -> Ground_Surface_Contact_Patch_Vx/4  "R2"
  Demux/571 -> Ground_Surface_Contact_Patch_Vx/3  "R1"
  Demux/570 -> Ground_Surface_Contact_Patch_Vx/2  "L2"
  Demux/569 -> Ground_Surface_Contact_Patch_Vx/1  "L1"
  Ground_Surface_Contact_Patch_Vx/1 -> Tire/12  "Ground_Surface_Contact_Patch_Vx"
  Demux/568 -> External_Friction_Scale_Factor/4  "R2"
  Demux/567 -> External_Friction_Scale_Factor/3  "R1"
  Demux/566 -> External_Friction_Scale_Factor/2  "L2"
  Demux/565 -> External_Friction_Scale_Factor/1  "L1"
  External_Friction_Scale_Factor/1 -> Tire/11  "External_Friction_Scale_Factor"
  Demux/564 -> Equivalent_Tread_Speed/4  "R2"
  Demux/563 -> Equivalent_Tread_Speed/3  "R1"
  Demux/562 -> Equivalent_Tread_Speed/2  "L2"
  Demux/561 -> Equivalent_Tread_Speed/1  "L1"
  Equivalent_Tread_Speed/1 -> Tire/10  "Equivalent_Tread_Speed"
  Demux/560 -> Effective_Rolling_Radius/4  "R2"
  Demux/559 -> Effective_Rolling_Radius/3  "R1"
  Demux/558 -> Effective_Rolling_Radius/2  "L2"
  Demux/557 -> Effective_Rolling_Radius/1  "L1"
  Effective_Rolling_Radius/1 -> Tire/9  "Effective_Rolling_Radius"
  Demux/556 -> Effective_Penetration/4  "R2"
  Demux/555 -> Effective_Penetration/3  "R1"
  Demux/554 -> Effective_Penetration/2  "L2"
  Demux/553 -> Effective_Penetration/1  "L1"
  Effective_Penetration/1 -> Tire/8  "Effective_Penetration"
  Demux/552 -> Effective_Closing_Speed/4  "R2"
  Demux/551 -> Effective_Closing_Speed/3  "R1"
  Demux/550 -> Effective_Closing_Speed/2  "L2"
  Demux/549 -> Effective_Closing_Speed/1  "L1"
  Effective_Closing_Speed/1 -> Tire/7  "Effective_Closing_Speed"
  Demux/548 -> Contact_Patch_Global_Z/4  "R2"
  Demux/547 -> Contact_Patch_Global_Z/3  "R1"
  Demux/546 -> Contact_Patch_Global_Z/2  "L2"
  Demux/545 -> Contact_Patch_Global_Z/1  "L1"
  Contact_Patch_Global_Z/1 -> Tire/6  "Contact_Patch_Global_Z"
  Demux/544 -> Contact_Patch_Global_Y/4  "R2"
  Demux/543 -> Contact_Patch_Global_Y/3  "R1"
  Demux/542 -> Contact_Patch_Global_Y/2  "L2"
  Demux/541 -> Contact_Patch_Global_Y/1  "L1"
  Contact_Patch_Global_Y/1 -> Tire/5  "Contact_Patch_Global_Y"
  Demux/540 -> Contact_Patch_Global_X/4  "R2"
  Demux/539 -> Contact_Patch_Global_X/3  "R1"
  Demux/538 -> Contact_Patch_Global_X/2  "L2"
  Demux/537 -> Contact_Patch_Global_X/1  "L1"
  Contact_Patch_Global_X/1 -> Tire/4  "Contact_Patch_Global_X"
  Demux/536 -> Contact_Patch_Global_dZdY/4  "R2"
  Demux/535 -> Contact_Patch_Global_dZdY/3  "R1"
  Demux/534 -> Contact_Patch_Global_dZdY/2  "L2"
  Demux/533 -> Contact_Patch_Global_dZdY/1  "L1"
  Contact_Patch_Global_dZdY/1 -> Tire/3  "Contact_Patch_Global_dZdY"
  Demux/532 -> Contact_Patch_Global_dZdX/4  "R2"
  Demux/531 -> Contact_Patch_Global_dZdX/3  "R1"
  Demux/530 -> Contact_Patch_Global_dZdX/2  "L2"
  Demux/529 -> Contact_Patch_Global_dZdX/1  "L1"
  Contact_Patch_Global_dZdX/1 -> Tire/2  "Contact_Patch_Global_dZdX"
  Demux/528 -> Actual_Tread_Speed/4  "R2"
  Demux/527 -> Actual_Tread_Speed/3  "R1"
  Demux/526 -> Actual_Tread_Speed/2  "L2"
  Demux/525 -> Actual_Tread_Speed/1  "L1"
  Actual_Tread_Speed/1 -> Tire/1  "Actual_Tread_Speed"
  Tire/1 -> OutputBus/55  "Tire"
  Demux/524 -> til_wheel_tire_rolling_states/9  "rolling_radius_twin_rear"
  Demux/523 -> til_wheel_tire_rolling_states/8  "rolling_radius_rear"
  Demux/522 -> til_wheel_tire_rolling_states/7  "rolling_radius_front"
  Demux/521 -> til_wheel_tire_rolling_states/6  "omega_free_twin_rear"
  Demux/520 -> til_wheel_tire_rolling_states/5  "omega_free_rear"
  Demux/519 -> til_wheel_tire_rolling_states/4  "omega_free_front"
  Demux/518 -> til_wheel_tire_rolling_states/3  "omega_actual_twin_rear"
  Demux/517 -> til_wheel_tire_rolling_states/2  "omega_actual_rear"
  Demux/516 -> til_wheel_tire_rolling_states/1  "omega_actual_front"
  til_wheel_tire_rolling_states/1 -> OutputBus/54  "til_wheel_tire_rolling_states"
  Demux/515 -> til_wheel_tire_kinematics/9  "longitudinal_slip_twin_rear"
  Demux/514 -> til_wheel_tire_kinematics/8  "longitudinal_slip_rear"
  Demux/513 -> til_wheel_tire_kinematics/7  "longitudinal_slip_front"
  Demux/512 -> til_wheel_tire_kinematics/6  "lateral_slip_twin_rear"
  Demux/511 -> til_wheel_tire_kinematics/5  "lateral_slip_rear"
  Demux/510 -> til_wheel_tire_kinematics/4  "lateral_slip_front"
  Demux/509 -> til_wheel_tire_kinematics/3  "inclination_angle_twin_rear"
  Demux/508 -> til_wheel_tire_kinematics/2  "inclination_angle_rear"
  Demux/507 -> til_wheel_tire_kinematics/1  "inclination_angle_front"
  til_wheel_tire_kinematics/1 -> OutputBus/53  "til_wheel_tire_kinematics"
  Demux/506 -> til_wheel_tire_forces/18  "rolling_resistance_twin_rear"
  Demux/505 -> til_wheel_tire_forces/17  "rolling_resistance_rear"
  Demux/504 -> til_wheel_tire_forces/16  "rolling_resistance_front"
  Demux/503 -> til_wheel_tire_forces/15  "overturning_moment_twin_rear"
  Demux/502 -> til_wheel_tire_forces/14  "overturning_moment_rear"
  Demux/501 -> til_wheel_tire_forces/13  "overturning_moment_front"
  Demux/500 -> til_wheel_tire_forces/12  "normal_twin_rear"
  Demux/499 -> til_wheel_tire_forces/11  "normal_rear"
  Demux/498 -> til_wheel_tire_forces/10  "normal_front"
  Demux/497 -> til_wheel_tire_forces/9  "longitudinal_twin_rear"
  Demux/496 -> til_wheel_tire_forces/8  "longitudinal_rear"
  Demux/495 -> til_wheel_tire_forces/7  "longitudinal_front"
  Demux/494 -> til_wheel_tire_forces/6  "lateral_twin_rear"
  Demux/493 -> til_wheel_tire_forces/5  "lateral_rear"
  Demux/492 -> til_wheel_tire_forces/4  "lateral_front"
  Demux/491 -> til_wheel_tire_forces/3  "aligning_torque_twin_rear"
  Demux/490 -> til_wheel_tire_forces/2  "aligning_torque_rear"
  Demux/489 -> til_wheel_tire_forces/1  "aligning_torque_front"
  til_wheel_tire_forces/1 -> OutputBus/52  "til_wheel_tire_forces"
  Demux/488 -> System_Mass_Center/13  "Tangential_Acceleration"
  Demux/487 -> System_Mass_Center/12  "Speed"
  Demux/486 -> System_Mass_Center/11  "Path_Curvature"
  Demux/485 -> System_Mass_Center/10  "Normal_Acceleration"
  Demux/484 -> System_Mass_Center/9  "Global_Z"
  Demux/483 -> System_Mass_Center/8  "Global_Y"
  Demux/482 -> System_Mass_Center/7  "Global_X"
  Demux/481 -> System_Mass_Center/6  "Global_Vz"
  Demux/480 -> System_Mass_Center/5  "Global_Vy"
  Demux/479 -> System_Mass_Center/4  "Global_Vx"
  Demux/478 -> System_Mass_Center/3  "Global_Az"
  Demux/477 -> System_Mass_Center/2  "Global_Ay"
  Demux/476 -> System_Mass_Center/1  "Global_Ax"
  System_Mass_Center/1 -> OutputBus/51  "System_Mass_Center"
  Demux/475 -> System/4  "Translational_Speed_Norm"
  Demux/474 -> System/3  "Translational_Acceleration_Norm"
  Demux/473 -> System/2  "Angular_Speed_Norm"
  Demux/472 -> System/1  "Angular_Acceleration_Norm"
  System/1 -> OutputBus/50  "System"
  Demux/471 -> Steering_Instant_Axis_Rotation/2  "R1"
  Demux/470 -> Steering_Instant_Axis_Rotation/1  "L1"
  Steering_Instant_Axis_Rotation/1 -> Suspension/14  "Steering_Instant_Axis_Rotation"
  Demux/469 -> Roll/2  "SUSP2"
  Demux/468 -> Roll/1  "SUSP1"
  Roll/1 -> Suspension/13  "Roll"
  Demux/467 -> Kingpin_Moment/1  "SUSP1"
  Kingpin_Moment/1 -> Suspension/12  "Kingpin_Moment"
  Demux/466 -> Jounce_Rate4/4  "R2"
  Demux/465 -> Jounce_Rate4/3  "R1"
  Demux/464 -> Jounce_Rate4/2  "L2"
  Demux/463 -> Jounce_Rate4/1  "L1"
  Jounce_Rate4/1 -> Suspension/11  "Jounce_Rate"
  Demux/462 -> Jounce_Acceleration4/4  "R2"
  Demux/461 -> Jounce_Acceleration4/3  "R1"
  Demux/460 -> Jounce_Acceleration4/2  "L2"
  Demux/459 -> Jounce_Acceleration4/1  "L1"
  Jounce_Acceleration4/1 -> Suspension/10  "Jounce_Acceleration"
  Demux/458 -> Jounce4/4  "R2"
  Demux/457 -> Jounce4/3  "R1"
  Demux/456 -> Jounce4/2  "L2"
  Demux/455 -> Jounce4/1  "L1"
  Jounce4/1 -> Suspension/9  "Jounce"
  Demux/454 -> Inst_Stiff_Force/4  "rear_right"
  Demux/453 -> Inst_Stiff_Force/3  "rear_left"
  Demux/452 -> Inst_Stiff_Force/2  "front_right"
  Demux/451 -> Inst_Stiff_Force/1  "front_left"
  Inst_Stiff_Force/1 -> Suspension/8  "Inst_Stiff_Force"
  Demux/450 -> Inst_Stiff_Deflection/4  "rear_right"
  Demux/449 -> Inst_Stiff_Deflection/3  "rear_left"
  Demux/448 -> Inst_Stiff_Deflection/2  "front_right"
  Demux/447 -> Inst_Stiff_Deflection/1  "front_left"
  Inst_Stiff_Deflection/1 -> Suspension/7  "Inst_Stiff_Deflection"
  Demux/446 -> base_velocity/4  "R2"
  Demux/445 -> base_velocity/3  "R1"
  Demux/444 -> base_velocity/2  "L2"
  Demux/443 -> base_velocity/1  "L1"
  base_velocity/1 -> Suspension/6  "base_velocity"
  Demux/442 -> base_deformation/4  "R2"
  Demux/441 -> base_deformation/3  "R1"
  Demux/440 -> base_deformation/2  "L2"
  Demux/439 -> base_deformation/1  "L1"
  base_deformation/1 -> Suspension/5  "base_deformation"
  Demux/438 -> base_acceleration/4  "R2"
  Demux/437 -> base_acceleration/3  "R1"
  Demux/436 -> base_acceleration/2  "L2"
  Demux/435 -> base_acceleration/1  "L1"
  base_acceleration/1 -> Suspension/4  "base_acceleration"
  Demux/434 -> Auxiliary_Roll_Force_at_element/2  "SUSP2"
  Demux/433 -> Auxiliary_Roll_Force_at_element/1  "SUSP1"
  Auxiliary_Roll_Force_at_element/1 -> Suspension/3  "Auxiliary_Roll_Force_at_element"
  Demux/432 -> Auxiliary_Roll_Force/4  "SUSP_R2"
  Demux/431 -> Auxiliary_Roll_Force/3  "SUSP_R1"
  Demux/430 -> Auxiliary_Roll_Force/2  "SUSP_L2"
  Demux/429 -> Auxiliary_Roll_Force/1  "SUSP_L1"
  Auxiliary_Roll_Force/1 -> Suspension/2  "Auxiliary_Roll_Force"
  Demux/428 -> Auxiliary_Roll_deformation_at_element/2  "SUSP2"
  Demux/427 -> Auxiliary_Roll_deformation_at_element/1  "SUSP1"
  Auxiliary_Roll_deformation_at_element/1 -> Suspension/1  "Auxiliary_Roll_deformation_at_element"
  Suspension/1 -> OutputBus/49  "Suspension"
  Demux/426 -> TieRod_Force_Right/3  "Z"
  Demux/425 -> TieRod_Force_Right/2  "Y"
  Demux/424 -> TieRod_Force_Right/1  "X"
  TieRod_Force_Right/1 -> Steering_System/6  "TieRod_Force_Right"
  Demux/423 -> TieRod_Force_Left/3  "Z"
  Demux/422 -> TieRod_Force_Left/2  "Y"
  Demux/421 -> TieRod_Force_Left/1  "X"
  TieRod_Force_Left/1 -> Steering_System/5  "TieRod_Force_Left"
  Demux/420 -> Steering_System/4  "Steering_Wheel_Torque"
  Demux/419 -> Steering_System/3  "Steering_column_deformation"
  Demux/418 -> Steering_System/2  "Rack_Force"
  Demux/417 -> Steering_System/1  "Rack_displacement"
  Steering_System/1 -> OutputBus/48  "Steering_System"
  Demux/416 -> PID_RH_At_Spring/4  "R2"
  Demux/415 -> PID_RH_At_Spring/3  "R1"
  Demux/414 -> PID_RH_At_Spring/2  "L2"
  Demux/413 -> PID_RH_At_Spring/1  "L1"
  PID_RH_At_Spring/1 -> Spring/10  "PID_RH_At_Spring"
  Demux/412 -> PID_PH_At_Spring/4  "R2"
  Demux/411 -> PID_PH_At_Spring/3  "R1"
  Demux/410 -> PID_PH_At_Spring/2  "L2"
  Demux/409 -> PID_PH_At_Spring/1  "L1"
  PID_PH_At_Spring/1 -> Spring/9  "PID_PH_At_Spring"
  Demux/408 -> PID_CW_At_Spring/4  "R2"
  Demux/407 -> PID_CW_At_Spring/3  "R1"
  Demux/406 -> PID_CW_At_Spring/2  "L2"
  Demux/405 -> PID_CW_At_Spring/1  "L1"
  PID_CW_At_Spring/1 -> Spring/8  "PID_CW_At_Spring"
  Demux/404 -> Jounce_Rate3/4  "R2"
  Demux/403 -> Jounce_Rate3/3  "R1"
  Demux/402 -> Jounce_Rate3/2  "L2"
  Demux/401 -> Jounce_Rate3/1  "L1"
  Jounce_Rate3/1 -> Spring/7  "Jounce_Rate"
  Demux/400 -> Jounce_Acceleration3/4  "R2"
  Demux/399 -> Jounce_Acceleration3/3  "R1"
  Demux/398 -> Jounce_Acceleration3/2  "L2"
  Demux/397 -> Jounce_Acceleration3/1  "L1"
  Jounce_Acceleration3/1 -> Spring/6  "Jounce_Acceleration"
  Demux/396 -> Jounce3/4  "R2"
  Demux/395 -> Jounce3/3  "R1"
  Demux/394 -> Jounce3/2  "L2"
  Demux/393 -> Jounce3/1  "L1"
  Jounce3/1 -> Spring/5  "Jounce"
  Demux/392 -> Force_Aux_At_Wheel/4  "R2"
  Demux/391 -> Force_Aux_At_Wheel/3  "R1"
  Demux/390 -> Force_Aux_At_Wheel/2  "L2"
  Demux/389 -> Force_Aux_At_Wheel/1  "L1"
  Force_Aux_At_Wheel/1 -> Spring/4  "Force_Aux_At_Wheel"
  Demux/388 -> Force_At_Wheel3/4  "R2"
  Demux/387 -> Force_At_Wheel3/3  "R1"
  Demux/386 -> Force_At_Wheel3/2  "L2"
  Demux/385 -> Force_At_Wheel3/1  "L1"
  Force_At_Wheel3/1 -> Spring/3  "Force_At_Wheel"
  Demux/384 -> Force_At_Spring/4  "R2"
  Demux/383 -> Force_At_Spring/3  "R1"
  Demux/382 -> Force_At_Spring/2  "L2"
  Demux/381 -> Force_At_Spring/1  "L1"
  Force_At_Spring/1 -> Spring/2  "Force_At_Spring"
  Demux/380 -> Aggregate_Force_At_Wheel/4  "R2"
  Demux/379 -> Aggregate_Force_At_Wheel/3  "R1"
  Demux/378 -> Aggregate_Force_At_Wheel/2  "L2"
  Demux/377 -> Aggregate_Force_At_Wheel/1  "L1"
  Aggregate_Force_At_Wheel/1 -> Spring/1  "Aggregate_Force_At_Wheel"
  Spring/1 -> OutputBus/47  "Spring"
  Demux/376 -> Sensor/16  "YawRate_gyro"
  Demux/375 -> Sensor/15  "Vz"
  Demux/374 -> Sensor/14  "Vy"
  Demux/373 -> Sensor/13  "Vx_gyro"
  Demux/372 -> Sensor/12  "Vx"
  Demux/371 -> Sensor/11  "Global_Z"
  Demux/370 -> Sensor/10  "Global_Y"
  Demux/369 -> Sensor/9  "Global_X"
  Demux/368 -> Sensor/8  "Az_Without_Gravity"
  Demux/367 -> Sensor/7  "Az"
  Demux/366 -> Sensor/6  "Ay_Without_Gravity"
  Demux/365 -> Sensor/5  "Ay"
  Demux/364 -> Sensor/4  "Ax_Without_Gravity"
  Demux/363 -> Sensor/3  "Ax"
  Demux/362 -> Sensor/2  "AccY_gyro"
  Demux/361 -> Sensor/1  "AccX_gyro"
  Sensor/1 -> OutputBus/46  "Sensor"
  Demux/360 -> rhs_rear_setup_sensor_data/1  "ride_height"
  rhs_rear_setup_sensor_data/1 -> OutputBus/45  "rhs_rear_setup_sensor_data"
  Demux/359 -> rhr_front_setup_sensor_data/1  "ride_height"
  rhr_front_setup_sensor_data/1 -> OutputBus/44  "rhr_front_setup_sensor_data"
  Demux/358 -> rhl_front_setup_sensor_data/1  "ride_height"
  rhl_front_setup_sensor_data/1 -> OutputBus/43  "rhl_front_setup_sensor_data"
  Demux/357 -> res_spr_rebound_stop_data/6  "velocity_rear"
  Demux/356 -> res_spr_rebound_stop_data/5  "velocity_front"
  Demux/355 -> res_spr_rebound_stop_data/4  "force_rear"
  Demux/354 -> res_spr_rebound_stop_data/3  "force_front"
  Demux/353 -> res_spr_rebound_stop_data/2  "displacement_rear"
  Demux/352 -> res_spr_rebound_stop_data/1  "displacement_front"
  res_spr_rebound_stop_data/1 -> OutputBus/42  "res_spr_rebound_stop_data"
  Demux/351 -> res_roll_dmp_rebound_stop_data/6  "velocity_rear"
  Demux/350 -> res_roll_dmp_rebound_stop_data/5  "velocity_front"
  Demux/349 -> res_roll_dmp_rebound_stop_data/4  "force_rear"
  Demux/348 -> res_roll_dmp_rebound_stop_data/3  "force_front"
  Demux/347 -> res_roll_dmp_rebound_stop_data/2  "displacement_rear"
  Demux/346 -> res_roll_dmp_rebound_stop_data/1  "displacement_front"
  res_roll_dmp_rebound_stop_data/1 -> OutputBus/41  "res_roll_dmp_rebound_stop_data"
  Demux/345 -> res_ins_rebound_stop_data/6  "velocity_rear"
  Demux/344 -> res_ins_rebound_stop_data/5  "velocity_front"
  Demux/343 -> res_ins_rebound_stop_data/4  "force_rear"
  Demux/342 -> res_ins_rebound_stop_data/3  "force_front"
  Demux/341 -> res_ins_rebound_stop_data/2  "displacement_rear"
  Demux/340 -> res_ins_rebound_stop_data/1  "displacement_front"
  res_ins_rebound_stop_data/1 -> OutputBus/40  "res_ins_rebound_stop_data"
  Demux/339 -> res_dmp_rebound_stop_data/6  "velocity_rear"
  Demux/338 -> res_dmp_rebound_stop_data/5  "velocity_front"
  Demux/337 -> res_dmp_rebound_stop_data/4  "force_rear"
  Demux/336 -> res_dmp_rebound_stop_data/3  "force_front"
  Demux/335 -> res_dmp_rebound_stop_data/2  "displacement_rear"
  Demux/334 -> res_dmp_rebound_stop_data/1  "displacement_front"
  res_dmp_rebound_stop_data/1 -> OutputBus/39  "res_dmp_rebound_stop_data"
  Demux/333 -> Jounce_Rate2/4  "R2"
  Demux/332 -> Jounce_Rate2/3  "R1"
  Demux/331 -> Jounce_Rate2/2  "L2"
  Demux/330 -> Jounce_Rate2/1  "L1"
  Jounce_Rate2/1 -> Rebound_Bumper/5  "Jounce_Rate"
  Demux/329 -> Jounce_Acceleration2/4  "R2"
  Demux/328 -> Jounce_Acceleration2/3  "R1"
  Demux/327 -> Jounce_Acceleration2/2  "L2"
  Demux/326 -> Jounce_Acceleration2/1  "L1"
  Jounce_Acceleration2/1 -> Rebound_Bumper/4  "Jounce_Acceleration"
  Demux/325 -> Jounce2/4  "R2"
  Demux/324 -> Jounce2/3  "R1"
  Demux/323 -> Jounce2/2  "L2"
  Demux/322 -> Jounce2/1  "L1"
  Jounce2/1 -> Rebound_Bumper/3  "Jounce"
  Demux/321 -> Force_At_Wheel2/4  "R2"
  Demux/320 -> Force_At_Wheel2/3  "R1"
  Demux/319 -> Force_At_Wheel2/2  "L2"
  Demux/318 -> Force_At_Wheel2/1  "L1"
  Force_At_Wheel2/1 -> Rebound_Bumper/2  "Force_At_Wheel"
  Demux/317 -> Force_At_Bumper1/4  "R2"
  Demux/316 -> Force_At_Bumper1/3  "R1"
  Demux/315 -> Force_At_Bumper1/2  "L2"
  Demux/314 -> Force_At_Bumper1/1  "L1"
  Force_At_Bumper1/1 -> Rebound_Bumper/1  "Force_At_Bumper"
  Rebound_Bumper/1 -> OutputBus/38  "Rebound_Bumper"
  Demux/313 -> nss_ride_spring_data/10  "velocity_rear"
  Demux/312 -> nss_ride_spring_data/9  "velocity_front"
  Demux/311 -> nss_ride_spring_data/8  "PID_PH_At_Spring_rear"
  Demux/310 -> nss_ride_spring_data/7  "PID_PH_At_Spring_front"
  Demux/309 -> nss_ride_spring_data/6  "force_rear"
  Demux/308 -> nss_ride_spring_data/5  "force_front"
  Demux/307 -> nss_ride_spring_data/4  "force_at_wheel_rear"
  Demux/306 -> nss_ride_spring_data/3  "force_at_wheel_front"
  Demux/305 -> nss_ride_spring_data/2  "displacement_rear"
  Demux/304 -> nss_ride_spring_data/1  "displacement_front"
  nss_ride_spring_data/1 -> OutputBus/37  "nss_ride_spring_data"
  Demux/303 -> nsr_ride_spring_data/6  "velocity_rear"
  Demux/302 -> nsr_ride_spring_data/5  "velocity_front"
  Demux/301 -> nsr_ride_spring_data/4  "force_rear"
  Demux/300 -> nsr_ride_spring_data/3  "force_front"
  Demux/299 -> nsr_ride_spring_data/2  "displacement_rear"
  Demux/298 -> nsr_ride_spring_data/1  "displacement_front"
  nsr_ride_spring_data/1 -> OutputBus/36  "nsr_ride_spring_data"
  Demux/297 -> nsl_ride_spring_data/6  "velocity_rear"
  Demux/296 -> nsl_ride_spring_data/5  "velocity_front"
  Demux/295 -> nsl_ride_spring_data/4  "force_rear"
  Demux/294 -> nsl_ride_spring_data/3  "force_front"
  Demux/293 -> nsl_ride_spring_data/2  "displacement_rear"
  Demux/292 -> nsl_ride_spring_data/1  "displacement_front"
  nsl_ride_spring_data/1 -> OutputBus/35  "nsl_ride_spring_data"
  Demux/291 -> Jounce_Rate1/4  "R2"
  Demux/290 -> Jounce_Rate1/3  "R1"
  Demux/289 -> Jounce_Rate1/2  "L2"
  Demux/288 -> Jounce_Rate1/1  "L1"
  Jounce_Rate1/1 -> Jounce_Bumper/5  "Jounce_Rate"
  Demux/287 -> Jounce_Acceleration1/4  "R2"
  Demux/286 -> Jounce_Acceleration1/3  "R1"
  Demux/285 -> Jounce_Acceleration1/2  "L2"
  Demux/284 -> Jounce_Acceleration1/1  "L1"
  Jounce_Acceleration1/1 -> Jounce_Bumper/4  "Jounce_Acceleration"
  Demux/283 -> Jounce1/4  "R2"
  Demux/282 -> Jounce1/3  "R1"
  Demux/281 -> Jounce1/2  "L2"
  Demux/280 -> Jounce1/1  "L1"
  Jounce1/1 -> Jounce_Bumper/3  "Jounce"
  Demux/279 -> Force_At_Wheel1/4  "R2"
  Demux/278 -> Force_At_Wheel1/3  "R1"
  Demux/277 -> Force_At_Wheel1/2  "L2"
  Demux/276 -> Force_At_Wheel1/1  "L1"
  Force_At_Wheel1/1 -> Jounce_Bumper/2  "Force_At_Wheel"
  Demux/275 -> Force_At_Bumper/4  "R2"
  Demux/274 -> Force_At_Bumper/3  "R1"
  Demux/273 -> Force_At_Bumper/2  "L2"
  Demux/272 -> Force_At_Bumper/1  "L1"
  Force_At_Bumper/1 -> Jounce_Bumper/1  "Force_At_Bumper"
  Jounce_Bumper/1 -> OutputBus/34  "Jounce_Bumper"
  Demux/271 -> jfs_torsional_stiffness_data/12  "Z_1"
  Demux/270 -> jfs_torsional_stiffness_data/11  "Y_1"
  Demux/269 -> jfs_torsional_stiffness_data/10  "X_1"
  Demux/268 -> jfs_torsional_stiffness_data/9  "TZ_1"
  Demux/267 -> jfs_torsional_stiffness_data/8  "TY_1"
  Demux/266 -> jfs_torsional_stiffness_data/7  "TX_1"
  Demux/265 -> jfs_torsional_stiffness_data/6  "FZ_1"
  Demux/264 -> jfs_torsional_stiffness_data/5  "FY_1"
  Demux/263 -> jfs_torsional_stiffness_data/4  "FX_1"
  Demux/262 -> jfs_torsional_stiffness_data/3  "AZ_1"
  Demux/261 -> jfs_torsional_stiffness_data/2  "AY_1"
  Demux/260 -> jfs_torsional_stiffness_data/1  "AX_1"
  jfs_torsional_stiffness_data/1 -> OutputBus/33  "jfs_torsional_stiffness_data"
  Demux/259 -> ins_inerter_data/10  "velocity_rear"
  Demux/258 -> ins_inerter_data/9  "velocity_front"
  Demux/257 -> ins_inerter_data/8  "force_rear"
  Demux/256 -> ins_inerter_data/7  "force_front"
  Demux/255 -> ins_inerter_data/6  "force_at_wheel_rear"
  Demux/254 -> ins_inerter_data/5  "force_at_wheel_front"
  Demux/253 -> ins_inerter_data/4  "displacement_rear"
  Demux/252 -> ins_inerter_data/3  "displacement_front"
  Demux/251 -> ins_inerter_data/2  "acceleration_rear"
  Demux/250 -> ins_inerter_data/1  "acceleration_front"
  ins_inerter_data/1 -> OutputBus/32  "ins_inerter_data"
  Demux/249 -> Hook_rear/18  "Local_Moment_Z"
  Demux/248 -> Hook_rear/17  "Local_Moment_Y"
  Demux/247 -> Hook_rear/16  "Local_Moment_X"
  Demux/246 -> Hook_rear/15  "Local_force_Z"
  Demux/245 -> Hook_rear/14  "Local_force_Y"
  Demux/244 -> Hook_rear/13  "Local_force_X"
  Demux/243 -> Hook_rear/12  "Hook_Z"
  Demux/242 -> Hook_rear/11  "Hook_Y"
  Demux/241 -> Hook_rear/10  "Hook_X"
  Demux/240 -> Hook_rear/9  "Hook_Theta"
  Demux/239 -> Hook_rear/8  "Hook_Psi"
  Demux/238 -> Hook_rear/7  "Hook_Phi"
  Demux/237 -> Hook_rear/6  "Global_Moment_Z"
  Demux/236 -> Hook_rear/5  "Global_Moment_Y"
  Demux/235 -> Hook_rear/4  "Global_Moment_X"
  Demux/234 -> Hook_rear/3  "Global_force_Z"
  Demux/233 -> Hook_rear/2  "Global_force_Y"
  Demux/232 -> Hook_rear/1  "Global_force_X"
  Hook_rear/1 -> OutputBus/31  "Hook_rear"
  Demux/231 -> Gyro/10  "sensor_3_Z"
  Demux/230 -> Gyro/9  "sensor_2_Z"
  Demux/229 -> Gyro/8  "sensor_1_Z"
  Demux/228 -> Gyro/7  "gyro_Y"
  Demux/227 -> Gyro/6  "gyro_X"
  Demux/226 -> Gyro/5  "gyro_VX"
  Demux/225 -> Gyro/4  "gyro_ACCY"
  Demux/224 -> Gyro/3  "gyro_ACCX"
  Demux/223 -> Gyro/2  "Driver_Z"
  Demux/222 -> Gyro/1  "Driver_X"
  Gyro/1 -> OutputBus/30  "Gyro"
  Demux/221 -> ges_chassis_XFORM/6  "Z"
  Demux/220 -> ges_chassis_XFORM/5  "Y"
  Demux/219 -> ges_chassis_XFORM/4  "X"
  Demux/218 -> ges_chassis_XFORM/3  "Theta"
  Demux/217 -> ges_chassis_XFORM/2  "Psi"
  Demux/216 -> ges_chassis_XFORM/1  "Phi"
  ges_chassis_XFORM/1 -> OutputBus/29  "ges_chassis_XFORM"
  Demux/215 -> fuel_consumption/4  "overall"
  Demux/214 -> fuel_consumption/3  "instantaneous_Liter_100km"
  Demux/213 -> fuel_consumption/2  "instantaneous"
  Demux/212 -> fuel_consumption/1  "BSFC"
  fuel_consumption/1 -> OutputBus/28  "fuel_consumption"
  Demux/211 -> engine/7  "torque"
  Demux/210 -> engine/6  "Power_KW"
  Demux/209 -> engine/5  "Power_HP"
  Demux/208 -> engine/4  "Min_engine_torque"
  Demux/207 -> engine/3  "Max_Engine_torque"
  Demux/206 -> engine/2  "engine_rpm"
  Demux/205 -> engine/1  "effective_throttle"
  engine/1 -> OutputBus/27  "engine"
  Demux/204 -> driving_machine_monitor/9  "target_vx"
  Demux/203 -> driving_machine_monitor/8  "target_ax"
  Demux/202 -> driving_machine_monitor/7  "path_z"
  Demux/201 -> driving_machine_monitor/6  "path_y"
  Demux/200 -> driving_machine_monitor/5  "path_x"
  Demux/199 -> driving_machine_monitor/4  "path_s"
  Demux/198 -> driving_machine_monitor/3  "path_distance"
  Demux/197 -> driving_machine_monitor/2  "path_curvature"
  Demux/196 -> driving_machine_monitor/1  "maneuver_ID"
  driving_machine_monitor/1 -> OutputBus/26  "driving_machine_monitor"
  Demux/195 -> driver_demands/7  "throttle"
  Demux/194 -> driver_demands/6  "steering_velocity"
  Demux/193 -> driver_demands/5  "steering"
  Demux/192 -> driver_demands/4  "gear"
  Demux/191 -> driver_demands/3  "clutch"
  Demux/190 -> driver_demands/2  "brake_pressure"
  Demux/189 -> driver_demands/1  "brake"
  driver_demands/1 -> OutputBus/25  "driver_demands"
  Demux/188 -> differential_torques/6  "output_torque_right_rear"
  Demux/187 -> differential_torques/5  "output_torque_right_front"
  Demux/186 -> differential_torques/4  "output_torque_left_rear"
  Demux/185 -> differential_torques/3  "output_torque_left_front"
  Demux/184 -> differential_torques/2  "differential_torque_rear"
  Demux/183 -> differential_torques/1  "differential_torque_front"
  differential_torques/1 -> OutputBus/24  "differential_torques"
  Demux/182 -> differential_speeds/6  "halfshaft_omega_right_rear"
  Demux/181 -> differential_speeds/5  "halfshaft_omega_right_front"
  Demux/180 -> differential_speeds/4  "halfshaft_omega_left_rear"
  Demux/179 -> differential_speeds/3  "halfshaft_omega_left_front"
  Demux/178 -> differential_speeds/2  "halfshaft_omega_delta_rear"
  Demux/177 -> differential_speeds/1  "halfshaft_omega_delta_front"
  differential_speeds/1 -> OutputBus/23  "differential_speeds"
  Demux/176 -> das_third_damper_data/6  "velocity_rear"
  Demux/175 -> das_third_damper_data/5  "velocity_front"
  Demux/174 -> das_third_damper_data/4  "force_rear"
  Demux/173 -> das_third_damper_data/3  "force_front"
  Demux/172 -> das_third_damper_data/2  "displacement_rear"
  Demux/171 -> das_third_damper_data/1  "displacement_front"
  das_third_damper_data/1 -> OutputBus/22  "das_third_damper_data"
  Demux/170 -> das_roll_damper_data/8  "velocity_rear"
  Demux/169 -> das_roll_damper_data/7  "velocity_front"
  Demux/168 -> das_roll_damper_data/6  "force_rear"
  Demux/167 -> das_roll_damper_data/5  "force_front"
  Demux/166 -> das_roll_damper_data/4  "force_at_wheel_rear"
  Demux/165 -> das_roll_damper_data/3  "force_at_wheel_front"
  Demux/164 -> das_roll_damper_data/2  "displacement_rear"
  Demux/163 -> das_roll_damper_data/1  "displacement_front"
  das_roll_damper_data/1 -> OutputBus/21  "das_roll_damper_data"
  Demux/162 -> das_ride_damper_data/6  "velocity_rear"
  Demux/161 -> das_ride_damper_data/5  "velocity_front"
  Demux/160 -> das_ride_damper_data/4  "force_rear"
  Demux/159 -> das_ride_damper_data/3  "force_front"
  Demux/158 -> das_ride_damper_data/2  "displacement_rear"
  Demux/157 -> das_ride_damper_data/1  "displacement_front"
  das_ride_damper_data/1 -> OutputBus/20  "das_ride_damper_data"
  Demux/156 -> dar_ride_damper_data/4  "velocity_rear"
  Demux/155 -> dar_ride_damper_data/3  "velocity_front"
  Demux/154 -> dar_ride_damper_data/2  "force_rear"
  Demux/153 -> dar_ride_damper_data/1  "force_front"
  dar_ride_damper_data/1 -> OutputBus/19  "dar_ride_damper_data"
  Demux/152 -> Jounce_Rate/4  "R2"
  Demux/151 -> Jounce_Rate/3  "R1"
  Demux/150 -> Jounce_Rate/2  "L2"
  Demux/149 -> Jounce_Rate/1  "L1"
  Jounce_Rate/1 -> Damper/5  "Jounce_Rate"
  Demux/148 -> Jounce_Acceleration/4  "R2"
  Demux/147 -> Jounce_Acceleration/3  "R1"
  Demux/146 -> Jounce_Acceleration/2  "L2"
  Demux/145 -> Jounce_Acceleration/1  "L1"
  Jounce_Acceleration/1 -> Damper/4  "Jounce_Acceleration"
  Demux/144 -> Jounce/4  "R2"
  Demux/143 -> Jounce/3  "R1"
  Demux/142 -> Jounce/2  "L2"
  Demux/141 -> Jounce/1  "L1"
  Jounce/1 -> Damper/3  "Jounce"
  Demux/140 -> Force_At_Wheel/4  "R2"
  Demux/139 -> Force_At_Wheel/3  "R1"
  Demux/138 -> Force_At_Wheel/2  "L2"
  Demux/137 -> Force_At_Wheel/1  "L1"
  Force_At_Wheel/1 -> Damper/2  "Force_At_Wheel"
  Demux/136 -> Force_At_Damper/4  "R2"
  Demux/135 -> Force_At_Damper/3  "R1"
  Demux/134 -> Force_At_Damper/2  "L2"
  Demux/133 -> Force_At_Damper/1  "L1"
  Force_At_Damper/1 -> Damper/1  "Force_At_Damper"
  Damper/1 -> OutputBus/18  "Damper"
  Demux/132 -> dal_ride_damper_data/4  "velocity_rear"
  Demux/131 -> dal_ride_damper_data/3  "velocity_front"
  Demux/130 -> dal_ride_damper_data/2  "force_rear"
  Demux/129 -> dal_ride_damper_data/1  "force_front"
  dal_ride_damper_data/1 -> OutputBus/17  "dal_ride_damper_data"
  Demux/128 -> cross_weight/4  "side_right_ratio"
  Demux/127 -> cross_weight/3  "nose_ratio"
  Demux/126 -> cross_weight/2  "crossR1L2_ratio"
  Demux/125 -> cross_weight/1  "crossL1R2_ratio"
  cross_weight/1 -> OutputBus/16  "cross_weight"
  Demux/124 -> condition_sensors/1  "side_slip_angle"
  condition_sensors/1 -> OutputBus/15  "condition_sensors"
  Demux/123 -> clutch/2  "torque"
  Demux/122 -> clutch/1  "slip_angle"
  clutch/1 -> OutputBus/14  "clutch"
  Demux/121 -> chassis_velocities/6  "yaw"
  Demux/120 -> chassis_velocities/5  "vertical"
  Demux/119 -> chassis_velocities/4  "roll"
  Demux/118 -> chassis_velocities/3  "pitch"
  Demux/117 -> chassis_velocities/2  "longitudinal"
  Demux/116 -> chassis_velocities/1  "lateral"
  chassis_velocities/1 -> OutputBus/13  "chassis_velocities"
  Demux/115 -> chassis_displacements/9  "yaw"
  Demux/114 -> chassis_displacements/8  "vertical_wrt_road"
  Demux/113 -> chassis_displacements/7  "vertical"
  Demux/112 -> chassis_displacements/6  "roll_wrt_road"
  Demux/111 -> chassis_displacements/5  "roll"
  Demux/110 -> chassis_displacements/4  "pitch_wrt_road"
  Demux/109 -> chassis_displacements/3  "pitch"
  Demux/108 -> chassis_displacements/2  "longitudinal"
  Demux/107 -> chassis_displacements/1  "lateral"
  chassis_displacements/1 -> OutputBus/12  "chassis_displacements"
  Demux/106 -> chassis_accelerations/6  "yaw"
  Demux/105 -> chassis_accelerations/5  "vertical"
  Demux/104 -> chassis_accelerations/4  "roll"
  Demux/103 -> chassis_accelerations/3  "pitch"
  Demux/102 -> chassis_accelerations/2  "longitudinal"
  Demux/101 -> chassis_accelerations/1  "lateral"
  chassis_accelerations/1 -> OutputBus/11  "chassis_accelerations"
  Demux/100 -> bus_spr_jounce_stop_data/6  "velocity_rear"
  Demux/99 -> bus_spr_jounce_stop_data/5  "velocity_front"
  Demux/98 -> bus_spr_jounce_stop_data/4  "force_rear"
  Demux/97 -> bus_spr_jounce_stop_data/3  "force_front"
  Demux/96 -> bus_spr_jounce_stop_data/2  "displacement_rear"
  Demux/95 -> bus_spr_jounce_stop_data/1  "displacement_front"
  bus_spr_jounce_stop_data/1 -> OutputBus/10  "bus_spr_jounce_stop_data"
  Demux/94 -> bus_roll_dmp_jounce_stop_data/6  "velocity_rear"
  Demux/93 -> bus_roll_dmp_jounce_stop_data/5  "velocity_front"
  Demux/92 -> bus_roll_dmp_jounce_stop_data/4  "force_rear"
  Demux/91 -> bus_roll_dmp_jounce_stop_data/3  "force_front"
  Demux/90 -> bus_roll_dmp_jounce_stop_data/2  "displacement_rear"
  Demux/89 -> bus_roll_dmp_jounce_stop_data/1  "displacement_front"
  bus_roll_dmp_jounce_stop_data/1 -> OutputBus/9  "bus_roll_dmp_jounce_stop_data"
  Demux/88 -> bus_ins_jounce_stop_data/6  "velocity_rear"
  Demux/87 -> bus_ins_jounce_stop_data/5  "velocity_front"
  Demux/86 -> bus_ins_jounce_stop_data/4  "force_rear"
  Demux/85 -> bus_ins_jounce_stop_data/3  "force_front"
  Demux/84 -> bus_ins_jounce_stop_data/2  "displacement_rear"
  Demux/83 -> bus_ins_jounce_stop_data/1  "displacement_front"
  bus_ins_jounce_stop_data/1 -> OutputBus/8  "bus_ins_jounce_stop_data"
  Demux/82 -> bus_dmp_jounce_stop_data/6  "velocity_rear"
  Demux/81 -> bus_dmp_jounce_stop_data/5  "velocity_front"
  Demux/80 -> bus_dmp_jounce_stop_data/4  "force_rear"
  Demux/79 -> bus_dmp_jounce_stop_data/3  "force_front"
  Demux/78 -> bus_dmp_jounce_stop_data/2  "displacement_rear"
  Demux/77 -> bus_dmp_jounce_stop_data/1  "displacement_front"
  bus_dmp_jounce_stop_data/1 -> OutputBus/7  "bus_dmp_jounce_stop_data"
  Demux/76 -> bur_rebound_stop_data/6  "velocity_rear"
  Demux/75 -> bur_rebound_stop_data/5  "velocity_front"
  Demux/74 -> bur_rebound_stop_data/4  "jounce_rear"
  Demux/73 -> bur_rebound_stop_data/3  "jounce_front"
  Demux/72 -> bur_rebound_stop_data/2  "force_rear"
  Demux/71 -> bur_rebound_stop_data/1  "force_front"
  bur_rebound_stop_data/1 -> OutputBus/6  "bur_rebound_stop_data"
  Demux/70 -> bur_jounce_stop_data/6  "velocity_rear"
  Demux/69 -> bur_jounce_stop_data/5  "velocity_front"
  Demux/68 -> bur_jounce_stop_data/4  "jounce_rear"
  Demux/67 -> bur_jounce_stop_data/3  "jounce_front"
  Demux/66 -> bur_jounce_stop_data/2  "force_rear"
  Demux/65 -> bur_jounce_stop_data/1  "force_front"
  bur_jounce_stop_data/1 -> OutputBus/5  "bur_jounce_stop_data"
  Demux/64 -> bul_rebound_stop_data/6  "velocity_rear"
  Demux/63 -> bul_rebound_stop_data/5  "velocity_front"
  Demux/62 -> bul_rebound_stop_data/4  "jounce_rear"
  Demux/61 -> bul_rebound_stop_data/3  "jounce_front"
  Demux/60 -> bul_rebound_stop_data/2  "force_rear"
  Demux/59 -> bul_rebound_stop_data/1  "force_front"
  bul_rebound_stop_data/1 -> OutputBus/4  "bul_rebound_stop_data"
  Demux/58 -> bul_jounce_stop_data/6  "velocity_rear"
  Demux/57 -> bul_jounce_stop_data/5  "velocity_front"
  Demux/56 -> bul_jounce_stop_data/4  "jounce_rear"
  Demux/55 -> bul_jounce_stop_data/3  "jounce_front"
  Demux/54 -> bul_jounce_stop_data/2  "force_rear"
  Demux/53 -> bul_jounce_stop_data/1  "force_front"
  bul_jounce_stop_data/1 -> OutputBus/3  "bul_jounce_stop_data"
  Demux/52 -> Lockup_Rotation/4  "R2"
  Demux/51 -> Lockup_Rotation/3  "R1"
  Demux/50 -> Lockup_Rotation/2  "L2"
  Demux/49 -> Lockup_Rotation/1  "L1"
  Lockup_Rotation/1 -> Brake/7  "Lockup_Rotation"
  Demux/48 -> Locked_Switch/4  "R2"
  Demux/47 -> Locked_Switch/3  "R1"
  Demux/46 -> Locked_Switch/2  "L2"
  Demux/45 -> Locked_Switch/1  "L1"
  Locked_Switch/1 -> Brake/6  "Locked_Switch"
  Demux/44 -> Locked_Spring_Moment/4  "R2"
  Demux/43 -> Locked_Spring_Moment/3  "R1"
  Demux/42 -> Locked_Spring_Moment/2  "L2"
  Demux/41 -> Locked_Spring_Moment/1  "L1"
  Locked_Spring_Moment/1 -> Brake/5  "Locked_Spring_Moment"
  Demux/40 -> Locked_Moment/4  "R2"
  Demux/39 -> Locked_Moment/3  "R1"
  Demux/38 -> Locked_Moment/2  "L2"
  Demux/37 -> Locked_Moment/1  "L1"
  Locked_Moment/1 -> Brake/4  "Locked_Moment"
  Demux/36 -> Locked_Damper_Moment/4  "R2"
  Demux/35 -> Locked_Damper_Moment/3  "R1"
  Demux/34 -> Locked_Damper_Moment/2  "L2"
  Demux/33 -> Locked_Damper_Moment/1  "L1"
  Locked_Damper_Moment/1 -> Brake/3  "Locked_Damper_Moment"
  Demux/32 -> Chamber_Pressure/4  "R2"
  Demux/31 -> Chamber_Pressure/3  "R1"
  Demux/30 -> Chamber_Pressure/2  "L2"
  Demux/29 -> Chamber_Pressure/1  "L1"
  Chamber_Pressure/1 -> Brake/2  "Chamber_Pressure"
  Demux/28 -> Brake_Moment/4  "R2"
  Demux/27 -> Brake_Moment/3  "R1"
  Demux/26 -> Brake_Moment/2  "L2"
  Demux/25 -> Brake_Moment/1  "L1"
  Brake_Moment/1 -> Brake/1  "Brake_Moment"
  Brake/1 -> OutputBus/2  "Brake"
  Demux/24 -> aero_forces/24  "yaw_torque"
  Demux/23 -> aero_forces/23  "vertical_velocity"
  Demux/22 -> aero_forces/22  "steer"
  Demux/21 -> aero_forces/21  "side_slip"
  Demux/20 -> aero_forces/20  "roll_torque"
  Demux/19 -> aero_forces/19  "roll"
  Demux/18 -> aero_forces/18  "rear_sideforce"
  Demux/17 -> aero_forces/17  "rear_downforce"
  Demux/16 -> aero_forces/16  "pitch"
  Demux/15 -> aero_forces/15  "longitudinal_velocity"
  Demux/14 -> aero_forces/14  "lateral_velocity"
  Demux/13 -> aero_forces/13  "height_rear"
  Demux/12 -> aero_forces/12  "height_front"
  Demux/11 -> aero_forces/11  "height_auxiliary"
  Demux/10 -> aero_forces/10  "front_sideforce"
  Demux/9 -> aero_forces/9  "front_downforce"
  Demux/8 -> aero_forces/8  "drag_torque"
  Demux/7 -> aero_forces/7  "drag_force_rear"
  Demux/6 -> aero_forces/6  "drag_force_front"
  Demux/5 -> aero_forces/5  "drag_force"
  Demux/4 -> aero_forces/4  "drag_arm"
  Demux/3 -> aero_forces/3  "center_sideforce"
  Demux/2 -> aero_forces/2  "center_downforce"
  Demux/1 -> aero_forces/1  "aero_balance"
  aero_forces/1 -> OutputBus/1  "aero_forces"
  OutputBus/1 -> Out/1  "OutputBus"
  In/1 -> Demux/1
